simulink model "sliding_car"  (R2017a)
settings: Solver=VariableStepAuto  StartTime=0.0  StopTime=tf  RelTol=1e-3
values from neighbouring files (symbols this model uses):
  a = double(perc*D)    [init_vars.m]
  Cp_1 = 0    [init_vars.m]
  Cp_2 = 0    [init_vars.m]
  Fz_1 = g*(mc/4 + mi)    [init_vars.m]
  Fz_2 = g*(mc/4 + mi)    [init_vars.m]
  mu_1 = 1e-3    (= 0.001)    [init_vars.m]
  mu_2 = 1e-3    (= 0.001)    [init_vars.m]
  x0 = double(subs([qs; ps], [sys.descrip.syms.'; delta_i],                   [sys.descrip.model_params.'; delta_i_num]))    [init_vars.m]    (also in sim_blockdiagram.m)
undefined symbols (not defined in the file or in its folder): g, Ic_33, Ii_11, Ii_21, Ii_22, Ii_31, Ii_32, Ii_33, Il_11, Il_21, Il_22, Il_31, Il_32, Il_33, Io_11, Io_21, Io_22, Io_31, Io_32, Io_33, Ir_11, Ir_21, Ir_22, Ir_31, Ir_32, Ir_33, L, Lc, mc, mi, ml, mo, mr, R, sys, w
(part 2 of 5)

== matlab function sliding_car/Vehicle/Steering automobile model/Auxiliary matrices/Q ==
  data: x input; qp input; u input; kappa_1 input; kappa_2 input; alpha_1 input; alpha_2 input; Ii_11 parameter; Ii_21 parameter; Ii_22 parameter; Ii_31 parameter; Ii_32 parameter; Ii_33 parameter; Il_11 parameter; Il_21 parameter; Il_22 parameter; Il_31 parameter; Il_32 parameter; Il_33 parameter; Io_11 parameter; Io_21 parameter; Io_22 parameter; Io_31 parameter; Io_32 parameter; Io_33 parameter; Ir_11 parameter; Ir_21 parameter; Ir_22 parameter; Ir_31 parameter; Ir_32 parameter; Ir_33 parameter; Lc parameter; mc parameter; mi parameter; ml parameter; mo parameter; mr parameter; L parameter; w parameter; Q output
function Q  = InputMatrix(x, qp, u, kappa_1, kappa_2, alpha_1, alpha_2, ...
                          Ii_11, Ii_21, Ii_22, Ii_31, Ii_32, Ii_33, ...
                          Il_11, Il_21, Il_22, Il_31, Il_32, Il_33, ...
                          Io_11, Io_21, Io_22, Io_31, Io_32, Io_33, ...
                          Ir_11, Ir_21, Ir_22, Ir_31, Ir_32, Ir_33, ...
                          Lc, mc, mi, ml, mo, mr, L, w)
    %INPUTMATRIX
    %    Q = INPUTMATRIX(II_11,II_21,II_22,II_31,II_32,II_33,IL_11,IL_21,IL_22,IL_31,IL_32,IL_33,IO_11,IO_21,IO_22,IO_31,IO_32,IO_33,IR_11,IR_21,IR_22,IR_31,IR_32,IR_33,L,LC,DELTA_I,DELTA_O,DELTAP_I,DELTAP_O,F_PHI_I,F_PHI_L,F_PHI_O,F_PHI_R,MC,MI,ML,MO,MR,PHI_I,PHI_L,PHI_O,PHI_R,PHIP_I,PHIP_L,PHIP_O,PHIP_R,THETAP,THETA,W)

    %    This function was generated by the Symbolic Math Toolbox version 7.2.
    %    16-Oct-2020 13:53:49

    x_pos =  x(1);
    y_pos =  x(2);
    theta =  x(3);

    delta_i = x(4);
    delta_o = x(5);

    phi_i = x(6);
    phi_l = x(7);
    phi_o = x(8);
    phi_r = x(9);
    
    p1 = x(10);
    p2 = x(11);
    p3 = x(12);
    
    xp = qp(1);
    yp = qp(2);
    thetap = qp(3);
    deltap_i = qp(4);
    deltap_o = qp(5);
    phip_i = qp(6);
    phip_o = qp(7);
    phip_r = qp(8);
    phip_l = qp(9);
    
    f_phi_i = u(1);
    f_phi_o = u(2);
    f_phi_r = u(3);
    f_phi_l = u(4);

    
    t2 = sin(theta);
    t3 = cos(theta);
    t4 = thetap.^2;
    t5 = deltap_i.^2;
    t6 = delta_i+theta;
    t7 = sin(t6);
    t8 = deltap_o.^2;
    t9 = delta_o+theta;
    t10 = sin(t9);
    t11 = phi_l+theta;
    t12 = cos(t11);
    t13 = phi_r+theta;
    t14 = cos(t13);
    t15 = phip_l.^2;
    t16 = sin(t11);
    t17 = phip_r.^2;
    t18 = sin(t13);
    t19 = theta.*2.0;
    t20 = delta_i.*2.0;
    t21 = phi_i+t19+t20;
    t22 = cos(t21);
    t23 = phip_i.^2;
    t24 = delta_o.*2.0;
    t25 = phi_o+t19+t24;
    t26 = cos(t25);
    t27 = phip_o.^2;
    t28 = sin(t21);
    t29 = sin(t25);
    t30 = phi_l-t19;
    t31 = cos(t30);
    t32 = phi_l+t19;
    t33 = cos(t32);
    t34 = phi_r-t19;
    t35 = cos(t34);
    t36 = phi_r+t19;
    t37 = cos(t36);
    t38 = phi_l-theta;
    t39 = cos(t38);
    t40 = phi_l.*3.0;
    t41 = t40+theta;
    t42 = cos(t41);
    t43 = phi_r-theta;
    t44 = cos(t43);
    t45 = phi_r.*3.0;
    t46 = t45+theta;
    t47 = cos(t46);
    t48 = delta_i+phi_i+theta;
    t49 = cos(t48);
    t50 = delta_o+phi_o+theta;
    t51 = cos(t50);
    t52 = sin(t30);
    t53 = sin(t32);
    t54 = phi_l.*2.0;
    t55 = t54+theta;
    t56 = sin(t38);
    t57 = sin(t41);
    t58 = sin(t34);
    t59 = sin(t36);
    t60 = phi_r.*2.0;
    t61 = t60+theta;
    t62 = sin(t43);
    t63 = sin(t46);
    t64 = phi_l.*4.0;
    t65 = t64+theta;
    t66 = sin(t65);
    t67 = phi_r.*4.0;
    t68 = t67+theta;
    t69 = sin(t68);
    t70 = sin(t48);
    t71 = sin(t50);
    t72 = -phi_i+t19+t20;
    t73 = cos(t72);
    t74 = phi_i.*2.0;
    t75 = t19+t20+t74;
    t76 = cos(t75);
    t77 = t19+t20-t74;
    t78 = cos(t77);
    t79 = phi_i.*3.0;
    t80 = t19+t20+t79;
    t81 = cos(t80);
    t82 = -phi_o+t19+t24;
    t83 = cos(t82);
    t84 = phi_o.*2.0;
    t85 = t19+t24+t84;
    t86 = cos(t85);
    t87 = t19+t24-t84;
    t88 = cos(t87);
    t89 = phi_o.*3.0;
    t90 = t19+t24+t89;
    t91 = cos(t90);
    t92 = phi_i.*4.0;
    t93 = t19+t20+t92;
    t94 = t19+t20-t79;
    t95 = sin(t77);
    t96 = sin(t75);
    t97 = t19+t20-t92;
    t98 = sin(t97);
    t99 = sin(t93);
    t100 = phi_o.*4.0;
    t101 = t19+t24+t100;
    t102 = t19+t24-t89;
    t103 = sin(t87);
    t104 = sin(t85);
    t105 = t19+t24-t100;
    t106 = sin(t105);
    t107 = sin(t101);
    t108 = cos(t94);
    t109 = cos(t93);
    t110 = cos(t102);
    t111 = cos(t101);
    t112 = sin(t72);
    t113 = sin(t94);
    t114 = sin(t80);
    t115 = sin(t82);
    t116 = sin(t102);
    t117 = sin(t90);
    t118 = sin(t19);
    t119 = t19+t20;
    t120 = sin(t119);
    t121 = t19+t24;
    t122 = sin(t121);
    t123 = -t19+t54;
    t124 = cos(t123);
    t125 = t19+t54;
    t126 = cos(t125);
    t127 = -t19+t60;
    t128 = cos(t127);
    t129 = t19+t60;
    t130 = cos(t129);
    t131 = t40-theta;
    t132 = cos(t131);
    t133 = -t19+t40;
    t134 = cos(t133);
    t135 = t19+t40;
    t136 = cos(t135);
    t137 = t45-theta;
    t138 = cos(t137);
    t139 = -t19+t45;
    t140 = cos(t139);
    t141 = t19+t45;
    t142 = cos(t141);
    t143 = delta_i-phi_i+theta;
    t144 = cos(t143);
    t145 = delta_i-t79+theta;
    t146 = cos(t145);
    t147 = delta_i+t79+theta;
    t148 = cos(t147);
    t149 = delta_o-phi_o+theta;
    t150 = cos(t149);
    t151 = delta_o-t89+theta;
    t152 = cos(t151);
    t153 = delta_o+t89+theta;
    t154 = cos(t153);
    t155 = delta_i-t92+theta;
    t156 = delta_i+t92+theta;
    t157 = sin(t155);
    t158 = sin(t156);
    t159 = delta_o-t100+theta;
    t160 = delta_o+t100+theta;
    t161 = sin(t159);
    t162 = sin(t160);
    t163 = cos(t155);
    t164 = cos(t156);
    t165 = cos(t159);
    t166 = cos(t160);
    t167 = t54-theta;
    t168 = sin(t123);
    t169 = sin(t125);
    t170 = sin(t131);
    t171 = sin(t133);
    t172 = sin(t135);
    t173 = t60-theta;
    t174 = sin(t127);
    t175 = sin(t129);
    t176 = sin(t137);
    t177 = sin(t139);
    t178 = sin(t141);
    t179 = t64-theta;
    t180 = -t19+t64;
    t181 = t19+t64;
    t182 = sin(t179);
    t183 = sin(t180);
    t184 = sin(t181);
    t185 = t67-theta;
    t186 = -t19+t67;
    t187 = t19+t67;
    t188 = sin(t185);
    t189 = sin(t186);
    t190 = sin(t187);
    t191 = sin(t143);
    t192 = sin(t145);
    t193 = sin(t147);
    t194 = delta_i-t74+theta;
    t195 = delta_i+t74+theta;
    t196 = sin(t149);
    t197 = sin(t151);
    t198 = sin(t153);
    t199 = delta_o-t84+theta;
    t200 = delta_o+t84+theta;
    t201 = cos(t65);
    t202 = cos(t68);
    t203 = cos(t97);
    t204 = cos(t105);
    t205 = sin(t74);
    t206 = sin(t92);
    t207 = sin(t84);
    t208 = sin(t100);
    t209 = cos(t74);
    t210 = cos(t92);
    t211 = cos(t84);
    t212 = cos(t100);
    t213 = sin(t54);
    t214 = sin(t64);
    t215 = sin(t60);
    t216 = sin(t67);
    t217 = cos(t179);
    t218 = cos(t180);
    t219 = cos(t181);
    t220 = cos(t185);
    t221 = cos(t186);
    t222 = cos(t187);
    t223 = Ii_11.*t5.*t7.*(1.0./8.0);
    t224 = Ii_11.*t4.*t7.*(1.0./8.0);
    t225 = Ii_21.*t5.*t22.*(1.0./8.0);
    t226 = Ii_21.*t22.*t23.*(1.0./2.0);
    t227 = Ii_31.*t22.*t23.*(1.0./8.0);
    t228 = Ii_32.*t5.*t28.*(3.0./8.0);
    t229 = Ii_21.*t4.*t22.*(1.0./8.0);
    t230 = Ii_11.*t23.*t28.*(1.0./1.6e1);
    t231 = Ii_32.*t23.*t28.*(1.0./2.0);
    t232 = Ii_33.*t23.*t28.*(3.0./1.6e1);
    t233 = Ii_32.*t4.*t28.*(3.0./8.0);
    t234 = Ii_21.*t5.*t49.*(1.0./8.0);
    t235 = Ii_21.*t4.*t49.*(1.0./8.0);
    t236 = Ii_11.*t23.*t70.*(1.0./8.0);
    t237 = Ii_21.*t5.*t73.*(1.0./8.0);
    t238 = Ii_31.*t5.*t109.*(1.0./1.6e1);
    t239 = Ii_21.*t23.*t73.*(1.0./2.0);
    t240 = Ii_21.*t23.*t78.*(1.0./2.0);
    t241 = Ii_21.*t23.*t76.*(1.0./2.0);
    t242 = Ii_31.*t23.*t78.*(1.0./4.0);
    t243 = Ii_31.*t23.*t108.*(3.0./8.0);
    t244 = Ii_22.*t5.*t95.*(1.0./8.0);
    t245 = Ii_22.*t5.*t96.*(1.0./8.0);
    t246 = Ii_32.*t5.*t113.*(1.0./8.0);
    t247 = Ii_33.*t5.*t98.*(1.0./3.2e1);
    t248 = Ii_33.*t5.*t99.*(1.0./3.2e1);
    t249 = Ii_21.*t4.*t73.*(1.0./8.0);
    t250 = Ii_31.*t4.*t78.*(1.0./8.0);
    t251 = Ii_31.*t4.*t109.*(1.0./1.6e1);
    t252 = Ii_11.*t23.*t112.*(1.0./1.6e1);
    t253 = Ii_11.*t23.*t95.*(1.0./8.0);
    t254 = Ii_11.*t23.*t96.*(1.0./8.0);
    t255 = Ii_11.*t23.*t113.*(3.0./1.6e1);
    t256 = Ii_11.*t23.*t114.*(3.0./1.6e1);
    t257 = Ii_32.*t23.*t96.*(1.0./2.0);
    t258 = Ii_33.*t23.*t112.*(3.0./1.6e1);
    t259 = Ii_22.*t4.*t95.*(1.0./8.0);
    t260 = Ii_22.*t4.*t96.*(1.0./8.0);
    t261 = Ii_32.*t4.*t113.*(1.0./8.0);
    t262 = Ii_33.*t4.*t98.*(1.0./3.2e1);
    t263 = Ii_33.*t4.*t99.*(1.0./3.2e1);
    t264 = Ii_11.*t5.*t120.*(1.0./1.6e1);
    t265 = Ii_33.*t5.*t120.*(3.0./1.6e1);
    t266 = Ii_21.*t5.*t144.*(1.0./8.0);
    t267 = Ii_31.*t5.*t164.*(1.0./8.0);
    t268 = Ii_11.*t23.*t120.*(1.0./4.0);
    t269 = Ii_33.*t23.*t120.*(1.0./4.0);
    t270 = cos(t194);
    t271 = Ii_21.*t23.*t270.*(1.0./2.0);
    t272 = cos(t195);
    t273 = Ii_21.*t23.*t272.*(1.0./2.0);
    t274 = Ii_31.*t23.*t144.*(1.0./4.0);
    t275 = Ii_31.*t23.*t146.*(3.0./4.0);
    t276 = Ii_11.*t4.*t120.*(1.0./1.6e1);
    t277 = Ii_33.*t4.*t120.*(3.0./1.6e1);
    t278 = Ii_32.*t5.*t191.*(1.0./8.0);
    t279 = Ii_32.*t5.*t192.*(1.0./8.0);
    t280 = Ii_33.*t5.*t157.*(1.0./1.6e1);
    t281 = Ii_33.*t5.*t158.*(1.0./1.6e1);
    t282 = Ii_21.*t4.*t144.*(1.0./8.0);
    t283 = Ii_31.*t4.*t164.*(1.0./8.0);
    t284 = Ii_11.*t23.*t191.*(1.0./8.0);
    t285 = Ii_11.*t23.*t192.*(3.0./8.0);
    t286 = Ii_11.*t23.*t193.*(3.0./8.0);
    t287 = sin(t194);
    t288 = sin(t195);
    t289 = Ii_32.*t23.*t288.*(1.0./2.0);
    t290 = Ii_32.*t4.*t191.*(1.0./8.0);
    t291 = Ii_32.*t4.*t192.*(1.0./8.0);
    t292 = Ii_33.*t4.*t157.*(1.0./1.6e1);
    t293 = Ii_33.*t4.*t158.*(1.0./1.6e1);
    t294 = Ii_11.*phip_i.*t157.*thetap.*(1.0./2.0);
    t295 = Ii_33.*phip_i.*t158.*thetap.*(1.0./2.0);
    t296 = Ii_11.*deltap_i.*t7.*thetap.*(1.0./4.0);
    t297 = Ii_21.*deltap_i.*phip_i.*t22.*(1.0./8.0);
    t298 = Ii_21.*deltap_i.*t22.*thetap.*(1.0./4.0);
    t299 = Ii_32.*deltap_i.*phip_i.*t28.*(3.0./8.0);
    t300 = Ii_21.*phip_i.*t22.*thetap.*(1.0./8.0);
    t301 = Ii_32.*deltap_i.*t28.*thetap.*(3.0./4.0);
    t302 = Ii_32.*phip_i.*t28.*thetap.*(3.0./8.0);
    t303 = Ii_21.*deltap_i.*phip_i.*t49.*(1.0./4.0);
    t304 = Ii_21.*deltap_i.*t49.*thetap.*(1.0./4.0);
    t305 = Ii_21.*phip_i.*t49.*thetap.*(1.0./4.0);
    t306 = Ii_21.*deltap_i.*phip_i.*t108.*(3.0./8.0);
    t307 = Ii_31.*deltap_i.*phip_i.*t203.*(1.0./4.0);
    t308 = Ii_31.*deltap_i.*phip_i.*t109.*(1.0./4.0);
    t309 = Ii_21.*deltap_i.*t73.*thetap.*(1.0./4.0);
    t310 = Ii_31.*deltap_i.*t78.*thetap.*(1.0./4.0);
    t311 = Ii_31.*deltap_i.*t109.*thetap.*(1.0./8.0);
    t312 = Ii_31.*deltap_i.*phip_i.*t209.*(1.0./2.0);
    t313 = Ii_31.*deltap_i.*phip_i.*t210.*(3.0./2.0);
    t314 = Ii_11.*deltap_i.*phip_i.*t98.*(1.0./8.0);
    t315 = Ii_22.*deltap_i.*phip_i.*t96.*(1.0./4.0);
    t316 = Ii_32.*deltap_i.*phip_i.*t112.*(3.0./8.0);
    t317 = Ii_33.*deltap_i.*phip_i.*t95.*(1.0./4.0);
    t318 = Ii_33.*deltap_i.*phip_i.*t99.*(1.0./8.0);
    t319 = Ii_21.*phip_i.*t108.*thetap.*(3.0./8.0);
    t320 = Ii_31.*phip_i.*t203.*thetap.*(1.0./4.0);
    t321 = Ii_31.*phip_i.*t109.*thetap.*(1.0./4.0);
    t322 = Ii_22.*deltap_i.*t95.*thetap.*(1.0./4.0);
    t323 = Ii_22.*deltap_i.*t96.*thetap.*(1.0./4.0);
    t324 = Ii_32.*deltap_i.*t113.*thetap.*(1.0./4.0);
    t325 = Ii_33.*deltap_i.*t98.*thetap.*(1.0./1.6e1);
    t326 = Ii_33.*deltap_i.*t99.*thetap.*(1.0./1.6e1);
    t327 = Ii_33.*deltap_i.*phip_i.*t205.*(1.0./2.0);
    t328 = Ii_33.*deltap_i.*phip_i.*t206.*(3.0./4.0);
    t329 = Ii_31.*phip_i.*t209.*thetap.*(1.0./2.0);
    t330 = Ii_31.*phip_i.*t210.*thetap.*(3.0./2.0);
    t331 = Ii_11.*phip_i.*t98.*thetap.*(1.0./8.0);
    t332 = Ii_22.*phip_i.*t96.*thetap.*(1.0./4.0);
    t333 = Ii_32.*phip_i.*t112.*thetap.*(3.0./8.0);
    t334 = Ii_33.*phip_i.*t95.*thetap.*(1.0./4.0);
    t335 = Ii_33.*phip_i.*t99.*thetap.*(1.0./8.0);
    t336 = Ii_33.*phip_i.*t205.*thetap.*(1.0./2.0);
    t337 = Ii_33.*phip_i.*t206.*thetap.*(3.0./4.0);
    t338 = Ii_21.*deltap_i.*phip_i.*t146.*(3.0./4.0);
    t339 = Ii_31.*deltap_i.*phip_i.*t163;
    t340 = Ii_31.*deltap_i.*phip_i.*t164;
    t341 = Ii_11.*deltap_i.*t120.*thetap.*(1.0./8.0);
    t342 = Ii_33.*deltap_i.*t120.*thetap.*(3.0./8.0);
    t343 = Ii_21.*deltap_i.*t144.*thetap.*(1.0./4.0);
    t344 = Ii_31.*deltap_i.*t164.*thetap.*(1.0./4.0);
    t345 = Ii_11.*deltap_i.*phip_i.*t157.*(1.0./2.0);
    t346 = Ii_33.*deltap_i.*phip_i.*t158.*(1.0./2.0);
    t347 = Ii_21.*phip_i.*t146.*thetap.*(3.0./4.0);
    t348 = Ii_31.*phip_i.*t163.*thetap;
    t349 = Ii_31.*phip_i.*t164.*thetap;
    t350 = Ii_32.*deltap_i.*t191.*thetap.*(1.0./4.0);
    t351 = Ii_32.*deltap_i.*t192.*thetap.*(1.0./4.0);
    t352 = Ii_33.*deltap_i.*t157.*thetap.*(1.0./8.0);
    t353 = Ii_33.*deltap_i.*t158.*thetap.*(1.0./8.0);
    t354 = Io_11.*t8.*t10.*(1.0./8.0);
    t355 = Io_11.*t4.*t10.*(1.0./8.0);
    t356 = Io_21.*t8.*t26.*(1.0./8.0);
    t357 = Io_21.*t26.*t27.*(1.0./2.0);
    t358 = Io_31.*t26.*t27.*(1.0./8.0);
    t359 = Io_32.*t8.*t29.*(3.0./8.0);
    t360 = Io_21.*t4.*t26.*(1.0./8.0);
    t361 = Io_11.*t27.*t29.*(1.0./1.6e1);
    t362 = Io_32.*t27.*t29.*(1.0./2.0);
    t363 = Io_33.*t27.*t29.*(3.0./1.6e1);
    t364 = Io_32.*t4.*t29.*(3.0./8.0);
    t365 = Io_21.*t8.*t51.*(1.0./8.0);
    t366 = Io_21.*t4.*t51.*(1.0./8.0);
    t367 = Io_11.*t27.*t71.*(1.0./8.0);
    t368 = Io_21.*t8.*t83.*(1.0./8.0);
    t369 = Io_31.*t8.*t111.*(1.0./1.6e1);
    t370 = Io_21.*t27.*t83.*(1.0./2.0);
    t371 = Io_21.*t27.*t88.*(1.0./2.0);
    t372 = Io_21.*t27.*t86.*(1.0./2.0);
    t373 = Io_31.*t27.*t88.*(1.0./4.0);
    t374 = Io_31.*t27.*t110.*(3.0./8.0);
    t375 = Io_22.*t8.*t103.*(1.0./8.0);
    t376 = Io_22.*t8.*t104.*(1.0./8.0);
    t377 = Io_32.*t8.*t116.*(1.0./8.0);
    t378 = Io_33.*t8.*t106.*(1.0./3.2e1);
    t379 = Io_33.*t8.*t107.*(1.0./3.2e1);
    t380 = Io_21.*t4.*t83.*(1.0./8.0);
    t381 = Io_31.*t4.*t88.*(1.0./8.0);
    t382 = Io_31.*t4.*t111.*(1.0./1.6e1);
    t383 = Io_11.*t27.*t115.*(1.0./1.6e1);
    t384 = Io_11.*t27.*t103.*(1.0./8.0);
    t385 = Io_11.*t27.*t104.*(1.0./8.0);
    t386 = Io_11.*t27.*t116.*(3.0./1.6e1);
    t387 = Io_11.*t27.*t117.*(3.0./1.6e1);
    t388 = Io_32.*t27.*t104.*(1.0./2.0);
    t389 = Io_33.*t27.*t115.*(3.0./1.6e1);
    t390 = Io_22.*t4.*t103.*(1.0./8.0);
    t391 = Io_22.*t4.*t104.*(1.0./8.0);
    t392 = Io_32.*t4.*t116.*(1.0./8.0);
    t393 = Io_33.*t4.*t106.*(1.0./3.2e1);
    t394 = Io_33.*t4.*t107.*(1.0./3.2e1);
    t395 = Io_11.*t8.*t122.*(1.0./1.6e1);
    t396 = Io_33.*t8.*t122.*(3.0./1.6e1);
    t397 = Io_21.*t8.*t150.*(1.0./8.0);
    t398 = Io_31.*t8.*t166.*(1.0./8.0);
    t399 = Io_11.*t27.*t122.*(1.0./4.0);
    t400 = Io_33.*t27.*t122.*(1.0./4.0);
    t401 = cos(t199);
    t402 = Io_21.*t27.*t401.*(1.0./2.0);
    t403 = cos(t200);
    t404 = Io_21.*t27.*t403.*(1.0./2.0);
    t405 = Io_31.*t27.*t150.*(1.0./4.0);
    t406 = Io_31.*t27.*t152.*(3.0./4.0);
    t407 = Io_11.*t4.*t122.*(1.0./1.6e1);
    t408 = Io_33.*t4.*t122.*(3.0./1.6e1);
    t409 = Io_32.*t8.*t196.*(1.0./8.0);
    t410 = Io_32.*t8.*t197.*(1.0./8.0);
    t411 = Io_33.*t8.*t161.*(1.0./1.6e1);
    t412 = Io_33.*t8.*t162.*(1.0./1.6e1);
    t413 = Io_21.*t4.*t150.*(1.0./8.0);
    t414 = Io_31.*t4.*t166.*(1.0./8.0);
    t415 = Io_11.*t27.*t196.*(1.0./8.0);
    t416 = Io_11.*t27.*t197.*(3.0./8.0);
    t417 = Io_11.*t27.*t198.*(3.0./8.0);
    t418 = sin(t199);
    t419 = sin(t200);
    t420 = Io_32.*t27.*t419.*(1.0./2.0);
    t421 = Io_32.*t4.*t196.*(1.0./8.0);
    t422 = Io_32.*t4.*t197.*(1.0./8.0);
    t423 = Io_33.*t4.*t161.*(1.0./1.6e1);
    t424 = Io_33.*t4.*t162.*(1.0./1.6e1);
    t425 = Io_11.*phip_o.*t161.*thetap.*(1.0./2.0);
    t426 = Io_33.*phip_o.*t162.*thetap.*(1.0./2.0);
    t427 = Io_11.*deltap_o.*t10.*thetap.*(1.0./4.0);
    t428 = Io_21.*deltap_o.*phip_o.*t26.*(1.0./8.0);
    t429 = Io_21.*deltap_o.*t26.*thetap.*(1.0./4.0);
    t430 = Io_32.*deltap_o.*phip_o.*t29.*(3.0./8.0);
    t431 = Io_21.*phip_o.*t26.*thetap.*(1.0./8.0);
    t432 = Io_32.*deltap_o.*t29.*thetap.*(3.0./4.0);
    t433 = Io_32.*phip_o.*t29.*thetap.*(3.0./8.0);
    t434 = Io_21.*deltap_o.*phip_o.*t51.*(1.0./4.0);
    t435 = Io_21.*deltap_o.*t51.*thetap.*(1.0./4.0);
    t436 = Io_21.*phip_o.*t51.*thetap.*(1.0./4.0);
    t437 = Io_21.*deltap_o.*phip_o.*t110.*(3.0./8.0);
    t438 = Io_31.*deltap_o.*phip_o.*t204.*(1.0./4.0);
    t439 = Io_31.*deltap_o.*phip_o.*t111.*(1.0./4.0);
    t440 = Io_21.*deltap_o.*t83.*thetap.*(1.0./4.0);
    t441 = Io_31.*deltap_o.*t88.*thetap.*(1.0./4.0);
    t442 = Io_31.*deltap_o.*t111.*thetap.*(1.0./8.0);
    t443 = Io_31.*deltap_o.*phip_o.*t211.*(1.0./2.0);
    t444 = Io_31.*deltap_o.*phip_o.*t212.*(3.0./2.0);
    t445 = Io_11.*deltap_o.*phip_o.*t106.*(1.0./8.0);
    t446 = Io_22.*deltap_o.*phip_o.*t104.*(1.0./4.0);
    t447 = Io_32.*deltap_o.*phip_o.*t115.*(3.0./8.0);
    t448 = Io_33.*deltap_o.*phip_o.*t103.*(1.0./4.0);
    t449 = Io_33.*deltap_o.*phip_o.*t107.*(1.0./8.0);
    t450 = Io_21.*phip_o.*t110.*thetap.*(3.0./8.0);
    t451 = Io_31.*phip_o.*t204.*thetap.*(1.0./4.0);
    t452 = Io_31.*phip_o.*t111.*thetap.*(1.0./4.0);
    t453 = Io_22.*deltap_o.*t103.*thetap.*(1.0./4.0);
    t454 = Io_22.*deltap_o.*t104.*thetap.*(1.0./4.0);
    t455 = Io_32.*deltap_o.*t116.*thetap.*(1.0./4.0);
    t456 = Io_33.*deltap_o.*t106.*thetap.*(1.0./1.6e1);
    t457 = Io_33.*deltap_o.*t107.*thetap.*(1.0./1.6e1);
    t458 = Io_33.*deltap_o.*phip_o.*t207.*(1.0./2.0);
    t459 = Io_33.*deltap_o.*phip_o.*t208.*(3.0./4.0);
    t460 = Io_31.*phip_o.*t211.*thetap.*(1.0./2.0);
    t461 = Io_31.*phip_o.*t212.*thetap.*(3.0./2.0);
    t462 = Io_11.*phip_o.*t106.*thetap.*(1.0./8.0);
    t463 = Io_22.*phip_o.*t104.*thetap.*(1.0./4.0);
    t464 = Io_32.*phip_o.*t115.*thetap.*(3.0./8.0);
    t465 = Io_33.*phip_o.*t103.*thetap.*(1.0./4.0);
    t466 = Io_33.*phip_o.*t107.*thetap.*(1.0./8.0);
    t467 = Io_33.*phip_o.*t207.*thetap.*(1.0./2.0);
    t468 = Io_33.*phip_o.*t208.*thetap.*(3.0./4.0);
    t469 = Io_21.*deltap_o.*phip_o.*t152.*(3.0./4.0);
    t470 = Io_31.*deltap_o.*phip_o.*t165;
    t471 = Io_31.*deltap_o.*phip_o.*t166;
    t472 = Io_11.*deltap_o.*t122.*thetap.*(1.0./8.0);
    t473 = Io_33.*deltap_o.*t122.*thetap.*(3.0./8.0);
    t474 = Io_21.*deltap_o.*t150.*thetap.*(1.0./4.0);
    t475 = Io_31.*deltap_o.*t166.*thetap.*(1.0./4.0);
    t476 = Io_11.*deltap_o.*phip_o.*t161.*(1.0./2.0);
    t477 = Io_33.*deltap_o.*phip_o.*t162.*(1.0./2.0);
    t478 = Io_21.*phip_o.*t152.*thetap.*(3.0./4.0);
    t479 = Io_31.*phip_o.*t165.*thetap;
    t480 = Io_31.*phip_o.*t166.*thetap;
    t481 = Io_32.*deltap_o.*t196.*thetap.*(1.0./4.0);
    t482 = Io_32.*deltap_o.*t197.*thetap.*(1.0./4.0);
    t483 = Io_33.*deltap_o.*t161.*thetap.*(1.0./8.0);
    t484 = Io_33.*deltap_o.*t162.*thetap.*(1.0./8.0);
    t485 = cos(delta_i);
    t486 = sin(delta_i);
    t487 = cos(t20);
    t488 = sin(t20);
    t489 = cos(t19);
    t490 = sin(phi_i);
    t491 = cos(phi_i);
    t492 = cos(t79);
    t493 = sin(t79);
    t494 = cos(delta_o);
    t495 = sin(delta_o);
    t496 = cos(t24);
    t497 = sin(t24);
    t498 = sin(phi_o);
    t499 = cos(phi_o);
    t500 = cos(t89);
    t501 = sin(t89);
    t502 = cos(phi_r);
    t503 = t502.^2;
    t504 = sin(phi_r);
    t505 = t504.^2;
    t506 = t2.^2;
    t507 = t503.^2;
    t508 = t3.^2;
    t509 = t505.^2;
    t510 = cos(phi_l);
    t511 = t510.^2;
    t512 = sin(phi_l);
    t513 = t512.^2;
    t514 = t511.^2;
    t515 = t513.^2;
    aux = t223+t224+t225+t226+t227+t228+t229+t230+t231+t232+t233+t234+t235+t236+t237+t238+t239+t240+t241+t242+t243+...
         t244+t245+t246+t247+t248+t249+t250+t251+t252+t253+t254+t255+t256+t257+t258+t259+t260+t261+t262+t263+t264+...
         t265+t266+t267+t268+t269+t271+t273+t274+t275+t276+t277+t278+t279+t280+t281+t282+t283+t284+t285+t286+t289+...
         t290+t291+t292+t293+t294+t295+t296+t297+t298+t299+t300+t301+t302+t303+t304+t305+t306+t307+t308+t309+t310+...
         t311+t312+t313+t314+t315+t316+t317+t318+t319+t320+t321+t322+t323+t324+t325+t326+t327+t328+t329+t330+t331+...
         t332+t333+t334+t335+t336+t337+t338+t339+t340+t341+t342+t343+t344+t345+t346+t347+t348+t349+t350+t351+t352+...
         t353+t354+t355+t356+t357+t358+t359+t360+t361+t362+t363+t364+t365+t366+t367+t368+t369+t370+t371+t372+t373+...
         t374+t375+t376+t377+t378+t379+t380+t381+t382+t383+t384+t385+t386+t387+t388+t389+t390+t391+t392+t393+t394+...
         t395+t396+t397+t398+t399+t400+t402+t404+t405+t406+t407+t408+t409+t410+t411+t412+t413+t414+t415+t416+t417+...
         t420+t421+t422+t423+t424+t425+t426+t427+t428+t429+t430+t431+t432+t433+t434+t435+t436+t437+t438+t439+t440+...
         t441+t442+t443+t444+t445+t446+t447+t448+t449+t450+t451+t452+t453+t454+t455+t456+t457+t458+t459+t460+t461+...
         t462+t463+t464+t465+t466+t467+t468+t469+t470+t471+t472+t473+t474+t475+t476+t477+t478+t479+t480+t481+t482;
     
    aux2 = t354+t355+t356+t357+t358+t359+t360+t361+t362+t363+t364+t365+t366+t367+t368+t369+t370+t371+t372+t373+t374+...
           t375+t376+t377+t378+t379+t380+t381+t382+t383+t384+t385+t386+t387+t388+t389+t390+t391+t392+t393+t394+t395+...
           t396+t397+t398+t399+t400+t402+t404+t405+t406+t407+t408+t409+t410+t411+t412+t413+t414+t415+t416+t417+t420+...
           t421+t422+t423+t424+t425+t426+t427+t428+t429+t430+t431+t432+t433+t434+t435+t436+t437+t438+t439+t440+t441+...
           t442+t443+t444+t445+t446+t447+t448+t449+t450+t451+t452+t453+t454+t455+t456+t457+t458+t459+t460+t461+t462+...
           t463+t464+t465+t466+t467+t468+t469+t470+t471+t472+t473+t474+t475+t476+t477+t478+t479+t480+t481+t482+t483+t484;
    
    aux3 = t223+t224+t225+t226+t227+t228+t229+t230+t231+t232+t233+t234+t235+t236+t237+t238+t239+t240+t241+t242+t243+...
           t244+t245+t246+t247+t248+t249+t250+t251+t252+t253+t254+t255+t256+t257+t258+t259+t260+t261+t262+t263+t264+...
           t265+t266+t267+t268+t269+t271+t273+t274+t275+t276+t277+t278+t279+t280+t281+t282+t283+t284+t285+t286+t289+t290+...
           t291+t292+t293+t294+t295+t296+t297+t298+t299+t300+t301+t302+t303+t304+t305+t306+t307+t308+t309+t310+t311+t312+...
           t313+t314+t315+t316+t317+t318+t319+t320+t321+t322+t323+t324+t325+t326+t327+t328+t329+t330+t331+t332+t333+...
           t334+t335+t336+t337+t338+t339+t340+t341+t342+t343+t344+t345+t346+t347+t348+t349+t350+t351+t352+t353;
    
    Q11 = t4.*(L.*mi.*t2.*2.0+L.*mo.*t2.*2.0+Lc.*mc.*t2.*2.0-mi.*t3.*w-ml.*t3.*w+mo.*t3.*w+mr.*t3.*w).*(-1.0./2.0);
    
    Q21 = t4.*(L.*mi.*t3.*2.0+L.*mo.*t3.*2.0+Lc.*mc.*t3.*2.0+mi.*t2.*w+ml.*t2.*w-mo.*t2.*w-mr.*t2.*w).*(1.0./2.0);
    
    Q31 = aux+t483+t484+Il_32.*t15.*sin(t55).*(1.0./2.0)+Il_32.*t15.*sin(t167).*(1.0./2.0)+Ir_32.*t17.*sin(t61).*(1.0./2.0)+...
         Ir_32.*t17.*sin(t173).*(1.0./2.0)-Ii_33.*t4.*t7.*(1.0./8.0)-Ii_33.*t5.*t7.*(1.0./8.0)-Ii_22.*t23.*t28.*(1.0./4.0)-...
         Ii_31.*t23.*t49.*(1.0./4.0)-Ii_21.*t4.*t81.*(1.0./8.0)-Ii_32.*t4.*t70.*(1.0./8.0)-Ii_21.*t5.*t81.*(1.0./8.0)-Ii_32.*t5.*t70.*(1.0./8.0)-...
         Ii_31.*t4.*t76.*(1.0./8.0)-Ii_31.*t5.*t76.*(1.0./8.0)-Ii_11.*t4.*t98.*(1.0./3.2e1)-Ii_11.*t4.*t99.*(1.0./3.2e1)-...
         Ii_11.*t5.*t98.*(1.0./3.2e1)-Ii_11.*t5.*t99.*(1.0./3.2e1)-Ii_33.*t23.*t70.*(1.0./8.0)-Ii_31.*t23.*t73.*(1.0./8.0)-...
         Ii_31.*t23.*t76.*(1.0./4.0)-Ii_33.*t4.*t95.*(1.0./8.0)-Ii_21.*t4.*t108.*(1.0./8.0)-Ii_33.*t4.*t96.*(1.0./8.0)-...
         Ii_33.*t5.*t95.*(1.0./8.0)-Ii_33.*t5.*t96.*(1.0./8.0)-Ii_31.*t23.*t81.*(3.0./8.0)-Ii_22.*t4.*t120.*(1.0./4.0)-...
         Ii_22.*t5.*t120.*(1.0./4.0)-Ii_32.*t4.*t112.*(3.0./8.0)-Ii_32.*t5.*t112.*(3.0./8.0)-Ii_32.*t4.*t114.*(1.0./8.0)-...
         Ii_32.*t23.*t95.*(1.0./2.0)-Ii_32.*t5.*t114.*(1.0./8.0)-Ii_33.*t23.*t95.*(1.0./8.0)-Ii_33.*t23.*t96.*(1.0./8.0)-...
         Ii_22.*t23.*t112.*(1.0./4.0)-Ii_22.*t23.*t120.*(1.0./2.0)-Ii_32.*t23.*t112.*(1.0./2.0)-Ii_33.*t23.*t113.*(3.0./1.6e1)-...
         Ii_33.*t23.*t114.*(3.0./1.6e1)-Ii_21.*t4.*t146.*(1.0./8.0)-Ii_11.*t4.*t157.*(1.0./1.6e1)-Ii_21.*t5.*t146.*(1.0./8.0)-...
         Ii_11.*t4.*t158.*(1.0./1.6e1)-Ii_11.*t5.*t157.*(1.0./1.6e1)-Ii_21.*t4.*t148.*(1.0./8.0)-Ii_11.*t5.*t158.*(1.0./1.6e1)-...
         Ii_21.*t5.*t148.*(1.0./8.0)-Ii_31.*t4.*t163.*(1.0./8.0)-Ii_31.*t5.*t163.*(1.0./8.0)-Ii_31.*t23.*t148.*(3.0./4.0)-Ii_32.*t4.*t193.*(1.0./8.0)-...
         Ii_32.*t5.*t193.*(1.0./8.0)-Ii_31.*t4.*t203.*(1.0./1.6e1)-Ii_33.*t23.*t191.*(1.0./8.0)-Ii_33.*t23.*t192.*(3.0./8.0)-Ii_33.*t23.*t193.*(3.0./8.0)-...
         Ii_32.*t23.*t287.*(1.0./2.0)+Il_11.*t2.*t4.*(1.0./8.0)+Il_21.*t4.*t12.*(1.0./8.0)-Il_33.*t2.*t4.*(1.0./8.0)+Il_11.*t15.*t16.*(1.0./8.0)-...
         Il_32.*t4.*t16.*(1.0./8.0)+Il_21.*t4.*t31.*(1.0./8.0)+Il_21.*t4.*t33.*(1.0./8.0)-Il_31.*t12.*t15.*(1.0./4.0)+Il_21.*t4.*t39.*(1.0./8.0)-Il_33.*t15.*t16.*(1.0./8.0)-...
         Il_21.*t4.*t42.*(1.0./8.0)+Il_21.*t15.*t31.*(1.0./2.0)+Il_21.*t15.*t33.*(1.0./2.0)-Il_31.*t15.*t31.*(1.0./8.0)-...
         Il_11.*t15.*t52.*(1.0./1.6e1)+Il_11.*t15.*t53.*(1.0./1.6e1)+Il_31.*t15.*t33.*(1.0./8.0)-Il_11.*t4.*t66.*(1.0./1.6e1)-...
         Il_11.*t15.*t56.*(1.0./8.0)+Il_11.*t15.*t57.*(3.0./8.0)+Il_31.*t15.*t39.*(1.0./4.0)-Il_31.*t15.*t42.*(3.0./4.0)+Il_32.*t4.*t52.*(3.0./8.0)+...
         Il_22.*t15.*t52.*(1.0./4.0)+Il_32.*t4.*t53.*(3.0./8.0)-Il_22.*t15.*t53.*(1.0./4.0)-Il_32.*t4.*t56.*(1.0./8.0)-Il_32.*t4.*t57.*(1.0./8.0)+...
         Il_32.*t15.*t52.*(1.0./2.0)+Il_32.*t15.*t53.*(1.0./2.0)-Il_33.*t15.*t52.*(3.0./1.6e1)+Il_33.*t15.*t53.*(3.0./1.6e1)+Il_33.*t4.*t66.*(1.0./1.6e1)+...
         Il_33.*t15.*t56.*(1.0./8.0)-Il_33.*t15.*t57.*(3.0./8.0)+Il_11.*t4.*t118.*(1.0./1.6e1)+Il_11.*t15.*t118.*(1.0./4.0)-Il_22.*t4.*t118.*(1.0./4.0)-...
         Il_22.*t15.*t118.*(1.0./2.0)+Il_33.*t4.*t118.*(3.0./1.6e1)-Il_21.*t4.*t132.*(1.0./8.0)-Il_21.*t4.*t134.*(1.0./8.0)+Il_31.*t4.*t124.*(1.0./8.0)+...
         Il_21.*t15.*t124.*(1.0./2.0)-Il_21.*t4.*t136.*(1.0./8.0)-Il_31.*t4.*t126.*(1.0./8.0)+Il_21.*t15.*t126.*(1.0./2.0)+Il_33.*t15.*t118.*(1.0./4.0)+...
         Il_31.*t15.*t124.*(1.0./4.0)-Il_31.*t15.*t126.*(1.0./4.0)+Il_31.*t15.*t132.*(3.0./4.0)+Il_31.*t15.*t134.*(3.0./8.0)-Il_31.*t15.*t136.*(3.0./8.0)-...
         Il_11.*t15.*t168.*(1.0./8.0)-Il_22.*t4.*t168.*(1.0./8.0)+Il_11.*t15.*t169.*(1.0./8.0)+Il_22.*t4.*t169.*(1.0./8.0)-Il_11.*t15.*t170.*(3.0./8.0)+...
         Il_11.*t4.*t182.*(1.0./1.6e1)-Il_11.*t15.*t171.*(3.0./1.6e1)+Il_11.*t4.*t183.*(1.0./3.2e1)+Il_11.*t15.*t172.*(3.0./1.6e1)-...
         Il_11.*t4.*t184.*(1.0./3.2e1)+Il_33.*t4.*t168.*(1.0./8.0)-Il_32.*t4.*t170.*(1.0./8.0)-Il_33.*t4.*t169.*(1.0./8.0)-Il_32.*t4.*t171.*(1.0./8.0)-...
         Il_32.*t4.*t172.*(1.0./8.0)+Il_32.*t15.*t168.*(1.0./2.0)+Il_32.*t15.*t169.*(1.0./2.0)+Il_33.*t15.*t168.*(1.0./8.0)-Il_33.*t15.*t169.*(1.0./8.0)+...
         Il_33.*t15.*t170.*(3.0./8.0)-Il_33.*t4.*t182.*(1.0./1.6e1)+Il_33.*t15.*t171.*(3.0./1.6e1)-Il_33.*t4.*t183.*(1.0./3.2e1)-Il_33.*t15.*t172.*(3.0./1.6e1)+...
         Il_33.*t4.*t184.*(1.0./3.2e1)+Il_31.*t4.*t201.*(1.0./8.0)-Il_31.*t4.*t217.*(1.0./8.0)-Il_31.*t4.*t218.*(1.0./1.6e1)+Il_31.*t4.*t219.*(1.0./1.6e1)-...
         Io_33.*t4.*t10.*(1.0./8.0)-Io_33.*t8.*t10.*(1.0./8.0)-Io_22.*t27.*t29.*(1.0./4.0)-Io_32.*t4.*t71.*(1.0./8.0)-Io_31.*t27.*t51.*(1.0./4.0)-...
         Io_32.*t8.*t71.*(1.0./8.0)-Io_21.*t4.*t91.*(1.0./8.0)-Io_21.*t8.*t91.*(1.0./8.0)-Io_11.*t4.*t106.*(1.0./3.2e1)-Io_31.*t4.*t86.*(1.0./8.0)-...
         Io_11.*t4.*t107.*(1.0./3.2e1)-Io_11.*t8.*t106.*(1.0./3.2e1)-Io_31.*t8.*t86.*(1.0./8.0)-Io_11.*t8.*t107.*(1.0./3.2e1)-Io_33.*t27.*t71.*(1.0./8.0)-...
         Io_21.*t4.*t110.*(1.0./8.0)-Io_33.*t4.*t103.*(1.0./8.0)-Io_31.*t27.*t83.*(1.0./8.0)-Io_33.*t4.*t104.*(1.0./8.0)-Io_31.*t27.*t86.*(1.0./4.0)-Io_33.*t8.*t103.*(1.0./8.0)-...
         Io_33.*t8.*t104.*(1.0./8.0)-Io_22.*t4.*t122.*(1.0./4.0)-Io_31.*t27.*t91.*(3.0./8.0)-Io_32.*t4.*t115.*(3.0./8.0)-Io_22.*t8.*t122.*(1.0./4.0)-...
         Io_32.*t4.*t117.*(1.0./8.0)-Io_32.*t8.*t115.*(3.0./8.0)-Io_32.*t8.*t117.*(1.0./8.0)-Io_32.*t27.*t103.*(1.0./2.0)-Io_33.*t27.*t103.*(1.0./8.0)-...
         Io_22.*t27.*t115.*(1.0./4.0)-Io_33.*t27.*t104.*(1.0./8.0)-Io_22.*t27.*t122.*(1.0./2.0)-Io_32.*t27.*t115.*(1.0./2.0)-Io_11.*t4.*t161.*(1.0./1.6e1)-...
         Io_33.*t27.*t116.*(3.0./1.6e1)-Io_11.*t4.*t162.*(1.0./1.6e1)-Io_21.*t4.*t152.*(1.0./8.0)-Io_33.*t27.*t117.*(3.0./1.6e1)-Io_21.*t4.*t154.*(1.0./8.0)-...
         Io_11.*t8.*t161.*(1.0./1.6e1)-Io_11.*t8.*t162.*(1.0./1.6e1)-Io_21.*t8.*t152.*(1.0./8.0)-Io_21.*t8.*t154.*(1.0./8.0)-Io_31.*t4.*t165.*(1.0./8.0)-...
         Io_31.*t8.*t165.*(1.0./8.0)-Io_31.*t27.*t154.*(3.0./4.0)-Io_32.*t4.*t198.*(1.0./8.0)-Io_32.*t8.*t198.*(1.0./8.0)-Io_31.*t4.*t204.*(1.0./1.6e1)-...
         Io_33.*t27.*t196.*(1.0./8.0)-Io_33.*t27.*t197.*(3.0./8.0)-Io_33.*t27.*t198.*(3.0./8.0)-Io_32.*t27.*t418.*(1.0./2.0)+Ir_11.*t2.*t4.*(1.0./8.0)+...
         Ir_21.*t4.*t14.*(1.0./8.0)-Ir_33.*t2.*t4.*(1.0./8.0)+Ir_11.*t17.*t18.*(1.0./8.0)-Ir_32.*t4.*t18.*(1.0./8.0)+Ir_21.*t4.*t35.*(1.0./8.0)+...
         Ir_21.*t4.*t37.*(1.0./8.0)-Ir_31.*t14.*t17.*(1.0./4.0)-Ir_33.*t17.*t18.*(1.0./8.0)+Ir_21.*t4.*t44.*(1.0./8.0)-Ir_21.*t4.*t47.*(1.0./8.0)+...
         Ir_21.*t17.*t35.*(1.0./2.0)+Ir_21.*t17.*t37.*(1.0./2.0)-Ir_31.*t17.*t35.*(1.0./8.0)-Ir_11.*t4.*t69.*(1.0./1.6e1)+Ir_31.*t17.*t37.*(1.0./8.0)-...
         Ir_11.*t17.*t58.*(1.0./1.6e1)+Ir_11.*t17.*t59.*(1.0./1.6e1)-Ir_11.*t17.*t62.*(1.0./8.0)+Ir_11.*t17.*t63.*(3.0./8.0)+Ir_31.*t17.*t44.*(1.0./4.0)+...
         Ir_32.*t4.*t58.*(3.0./8.0)-Ir_31.*t17.*t47.*(3.0./4.0)+Ir_32.*t4.*t59.*(3.0./8.0)+Ir_22.*t17.*t58.*(1.0./4.0)-Ir_22.*t17.*t59.*(1.0./4.0)-...
         Ir_32.*t4.*t62.*(1.0./8.0)-Ir_32.*t4.*t63.*(1.0./8.0)+Ir_33.*t4.*t69.*(1.0./1.6e1)+Ir_32.*t17.*t58.*(1.0./2.0)+Ir_32.*t17.*t59.*(1.0./2.0)-...
         Ir_33.*t17.*t58.*(3.0./1.6e1)+Ir_33.*t17.*t59.*(3.0./1.6e1)+Ir_33.*t17.*t62.*(1.0./8.0)-Ir_33.*t17.*t63.*(3.0./8.0)+Ir_11.*t4.*t118.*(1.0./1.6e1)-...
         Ir_22.*t4.*t118.*(1.0./4.0)+Ir_11.*t17.*t118.*(1.0./4.0)+Ir_33.*t4.*t118.*(3.0./1.6e1)-Ir_22.*t17.*t118.*(1.0./2.0)-Ir_21.*t4.*t138.*(1.0./8.0)+...
         Ir_31.*t4.*t128.*(1.0./8.0)-Ir_21.*t4.*t140.*(1.0./8.0)-Ir_31.*t4.*t130.*(1.0./8.0)+Ir_21.*t17.*t128.*(1.0./2.0)-Ir_21.*t4.*t142.*(1.0./8.0)+...
         Ir_21.*t17.*t130.*(1.0./2.0)+Ir_33.*t17.*t118.*(1.0./4.0)+Ir_31.*t17.*t128.*(1.0./4.0)-Ir_31.*t17.*t130.*(1.0./4.0)+Ir_31.*t17.*t138.*(3.0./4.0)+...
         Ir_31.*t17.*t140.*(3.0./8.0)-Ir_31.*t17.*t142.*(3.0./8.0)-Ir_22.*t4.*t174.*(1.0./8.0)+Ir_22.*t4.*t175.*(1.0./8.0)-Ir_11.*t17.*t174.*(1.0./8.0)+...
         Ir_11.*t4.*t188.*(1.0./1.6e1)+Ir_11.*t17.*t175.*(1.0./8.0)+Ir_11.*t4.*t189.*(1.0./3.2e1)-Ir_11.*t17.*t176.*(3.0./8.0)-Ir_11.*t4.*t190.*(1.0./3.2e1)-...
         Ir_11.*t17.*t177.*(3.0./1.6e1)+Ir_11.*t17.*t178.*(3.0./1.6e1)+Ir_33.*t4.*t174.*(1.0./8.0)-Ir_32.*t4.*t176.*(1.0./8.0)-Ir_33.*t4.*t175.*(1.0./8.0)-...
         Ir_32.*t4.*t177.*(1.0./8.0)-Ir_32.*t4.*t178.*(1.0./8.0)+Ir_32.*t17.*t174.*(1.0./2.0)+Ir_32.*t17.*t175.*(1.0./2.0)+Ir_33.*t17.*t174.*(1.0./8.0)-...
         Ir_33.*t4.*t188.*(1.0./1.6e1)-Ir_33.*t17.*t175.*(1.0./8.0)-Ir_33.*t4.*t189.*(1.0./3.2e1)+Ir_33.*t17.*t176.*(3.0./8.0)+Ir_33.*t4.*t190.*(1.0./3.2e1)+...
         Ir_33.*t17.*t177.*(3.0./1.6e1)-Ir_33.*t17.*t178.*(3.0./1.6e1)+Ir_31.*t4.*t202.*(1.0./8.0)-Ir_31.*t4.*t220.*(1.0./8.0)-Ir_31.*t4.*t221.*(1.0./1.6e1)+...
         Ir_31.*t4.*t222.*(1.0./1.6e1)-Ii_21.*t5.*cos(phi_i.*-3.0+t19+t20).*(1.0./8.0)+Ii_31.*t5.*cos(phi_i.*-2.0+t19+t20).*(1.0./8.0)-Ii_31.*t5.*cos(phi_i.*-4.0+...
         t19+t20).*(1.0./1.6e1)-Io_21.*t8.*cos(phi_o.*-3.0+t19+t24).*(1.0./8.0)+Io_31.*t8.*cos(phi_o.*-2.0+t19+t24).*(1.0./8.0)-Io_31.*t8.*cos(phi_o.*-4.0+t19+...
         t24).*(1.0./1.6e1)+Il_21.*t15.*cos(t55).*(1.0./2.0)+Il_21.*t15.*cos(t167).*(1.0./2.0)+Ir_21.*t17.*cos(t61).*(1.0./2.0)+Ir_21.*t17.*cos(t173).*(1.0./2.0)-...
         Ii_21.*phip_i.*t73.*thetap.*(1.0./8.0)-Ii_21.*phip_i.*t81.*thetap.*(3.0./8.0)-Ii_32.*phip_i.*t70.*thetap.*(1.0./4.0)-Ii_31.*phip_i.*t76.*thetap.*(1.0./4.0)-...
         Ii_31.*phip_i.*t78.*thetap.*(1.0./4.0)-Ii_11.*phip_i.*t99.*thetap.*(1.0./8.0)-Ii_22.*phip_i.*t95.*thetap.*(1.0./4.0)-Ii_33.*phip_i.*t96.*thetap.*(1.0./4.0)-...
         Ii_33.*phip_i.*t98.*thetap.*(1.0./8.0)-Ii_32.*phip_i.*t113.*thetap.*(3.0./8.0)-Ii_32.*phip_i.*t114.*thetap.*(3.0./8.0)-Ii_21.*phip_i.*t144.*thetap.*(1.0./4.0)-...
         Ii_11.*phip_i.*t158.*thetap.*(1.0./2.0)-Ii_21.*phip_i.*t148.*thetap.*(3.0./4.0)-Ii_33.*phip_i.*t157.*thetap.*(1.0./2.0)-Ii_11.*phip_i.*t206.*thetap.*(3.0./4.0)-...
         Ii_32.*phip_i.*t191.*thetap.*(1.0./4.0)-Ii_32.*phip_i.*t192.*thetap.*(3.0./4.0)-Ii_32.*phip_i.*t193.*thetap.*(3.0./4.0)-Ii_22.*phip_i.*t205.*thetap.*(1.0./2.0)+...
         Il_21.*phip_l.*t12.*thetap.*(1.0./4.0)-Il_32.*phip_l.*t16.*thetap.*(1.0./4.0)-Il_21.*phip_l.*t31.*thetap.*(1.0./8.0)+Il_21.*phip_l.*t33.*thetap.*(1.0./8.0)-...
         Il_21.*phip_l.*t39.*thetap.*(1.0./4.0)-Il_21.*phip_l.*t42.*thetap.*(3.0./4.0)-Il_11.*phip_l.*t66.*thetap.*(1.0./2.0)-Il_32.*phip_l.*t52.*thetap.*(3.0./8.0)+...
         Il_32.*phip_l.*t53.*thetap.*(3.0./8.0)+Il_32.*phip_l.*t56.*thetap.*(1.0./4.0)-Il_32.*phip_l.*t57.*thetap.*(3.0./4.0)+Il_33.*phip_l.*t66.*thetap.*(1.0./2.0)+...
         Il_21.*phip_l.*t132.*thetap.*(3.0./4.0)+Il_21.*phip_l.*t134.*thetap.*(3.0./8.0)-Il_31.*phip_l.*t124.*thetap.*(1.0./4.0)-Il_21.*phip_l.*t136.*thetap.*(3.0./8.0)-...
         Il_31.*phip_l.*t126.*thetap.*(1.0./4.0)+Il_22.*phip_l.*t168.*thetap.*(1.0./4.0)+Il_22.*phip_l.*t169.*thetap.*(1.0./4.0)-Il_11.*phip_l.*t182.*thetap.*(1.0./2.0)-...
         Il_11.*phip_l.*t183.*thetap.*(1.0./8.0)-Il_11.*phip_l.*t184.*thetap.*(1.0./8.0)-Il_33.*phip_l.*t168.*thetap.*(1.0./4.0)+Il_32.*phip_l.*t170.*thetap.*(3.0./4.0)-...
         Il_33.*phip_l.*t169.*thetap.*(1.0./4.0)+Il_32.*phip_l.*t171.*thetap.*(3.0./8.0)-Il_32.*phip_l.*t172.*thetap.*(3.0./8.0)+Il_33.*phip_l.*t182.*thetap.*(1.0./2.0)+...
         Il_33.*phip_l.*t183.*thetap.*(1.0./8.0)+Il_33.*phip_l.*t184.*thetap.*(1.0./8.0)-Il_11.*phip_l.*t214.*thetap.*(3.0./4.0)+Il_31.*phip_l.*t201.*thetap-...
         Il_22.*phip_l.*t213.*thetap.*(1.0./2.0)+Il_33.*phip_l.*t213.*thetap.*(1.0./2.0)+Il_33.*phip_l.*t214.*thetap.*(3.0./4.0)+Il_31.*phip_l.*t217.*thetap+...
         Il_31.*phip_l.*t218.*thetap.*(1.0./4.0)+Il_31.*phip_l.*t219.*thetap.*(1.0./4.0)-Io_32.*phip_o.*t71.*thetap.*(1.0./4.0)-Io_21.*phip_o.*t83.*thetap.*(1.0./8.0)-...
         Io_21.*phip_o.*t91.*thetap.*(3.0./8.0)-Io_31.*phip_o.*t86.*thetap.*(1.0./4.0)-Io_11.*phip_o.*t107.*thetap.*(1.0./8.0)-Io_31.*phip_o.*t88.*thetap.*(1.0./4.0)-...
         Io_22.*phip_o.*t103.*thetap.*(1.0./4.0)-Io_33.*phip_o.*t104.*thetap.*(1.0./4.0)-Io_33.*phip_o.*t106.*thetap.*(1.0./8.0)-Io_32.*phip_o.*t116.*thetap.*(3.0./8.0)-...
         Io_32.*phip_o.*t117.*thetap.*(3.0./8.0)-Io_21.*phip_o.*t150.*thetap.*(1.0./4.0)-Io_11.*phip_o.*t162.*thetap.*(1.0./2.0)-Io_21.*phip_o.*t154.*thetap.*(3.0./4.0)-...
         Io_33.*phip_o.*t161.*thetap.*(1.0./2.0)-Io_11.*phip_o.*t208.*thetap.*(3.0./4.0)-Io_32.*phip_o.*t196.*thetap.*(1.0./4.0)-Io_22.*phip_o.*t207.*thetap.*(1.0./2.0)-...
         Io_32.*phip_o.*t197.*thetap.*(3.0./4.0)-Io_32.*phip_o.*t198.*thetap.*(3.0./4.0)+Ir_21.*phip_r.*t14.*thetap.*(1.0./4.0)-Ir_32.*phip_r.*t18.*thetap.*(1.0./4.0)-...
         Ir_21.*phip_r.*t35.*thetap.*(1.0./8.0)+Ir_21.*phip_r.*t37.*thetap.*(1.0./8.0)-Ir_21.*phip_r.*t44.*thetap.*(1.0./4.0)-Ir_21.*phip_r.*t47.*thetap.*(3.0./4.0)-...
         Ir_11.*phip_r.*t69.*thetap.*(1.0./2.0)-Ir_32.*phip_r.*t58.*thetap.*(3.0./8.0)+Ir_32.*phip_r.*t59.*thetap.*(3.0./8.0)+Ir_32.*phip_r.*t62.*thetap.*(1.0./4.0)-...
         Ir_32.*phip_r.*t63.*thetap.*(3.0./4.0)+Ir_33.*phip_r.*t69.*thetap.*(1.0./2.0)+Ir_21.*phip_r.*t138.*thetap.*(3.0./4.0)-Ir_31.*phip_r.*t128.*thetap.*(1.0./4.0)+...
         Ir_21.*phip_r.*t140.*thetap.*(3.0./8.0)-Ir_31.*phip_r.*t130.*thetap.*(1.0./4.0)-Ir_21.*phip_r.*t142.*thetap.*(3.0./8.0)+Ir_22.*phip_r.*t174.*thetap.*(1.0./4.0)+...
         Ir_22.*phip_r.*t175.*thetap.*(1.0./4.0)-Ir_11.*phip_r.*t188.*thetap.*(1.0./2.0)-Ir_11.*phip_r.*t189.*thetap.*(1.0./8.0)-Ir_11.*phip_r.*t190.*thetap.*(1.0./8.0)-...
         Ir_33.*phip_r.*t174.*thetap.*(1.0./4.0)+Ir_32.*phip_r.*t176.*thetap.*(3.0./4.0)-Ir_33.*phip_r.*t175.*thetap.*(1.0./4.0)+Ir_32.*phip_r.*t177.*thetap.*(3.0./8.0)-...
         Ir_32.*phip_r.*t178.*thetap.*(3.0./8.0)+Ir_33.*phip_r.*t188.*thetap.*(1.0./2.0)+Ir_33.*phip_r.*t189.*thetap.*(1.0./8.0)+Ir_33.*phip_r.*t190.*thetap.*(1.0./8.0)-...
         Ir_11.*phip_r.*t216.*thetap.*(3.0./4.0)+Ir_31.*phip_r.*t202.*thetap-Ir_22.*phip_r.*t215.*thetap.*(1.0./2.0)+Ir_33.*phip_r.*t215.*thetap.*(1.0./2.0)+...
         Ir_33.*phip_r.*t216.*thetap.*(3.0./4.0)+Ir_31.*phip_r.*t220.*thetap+Ir_31.*phip_r.*t221.*thetap.*(1.0./4.0)+Ir_31.*phip_r.*t222.*thetap.*(1.0./4.0)+...
         Il_31.*phip_l.*thetap.*cos(t54).*(1.0./2.0)+Il_31.*phip_l.*thetap.*cos(t64).*(3.0./2.0)+Ir_31.*phip_r.*thetap.*cos(t60).*(1.0./2.0)+Ir_31.*phip_r.*thetap.*cos(t67).*(3.0./2.0)-...
         Ii_21.*deltap_i.*phip_i.*t73.*(1.0./8.0)-Ii_21.*deltap_i.*phip_i.*t81.*(3.0./8.0)-Ii_32.*deltap_i.*phip_i.*t70.*(1.0./4.0)-Ii_31.*deltap_i.*phip_i.*t76.*(1.0./4.0)-...
         Ii_31.*deltap_i.*phip_i.*t78.*(1.0./4.0)-Ii_11.*deltap_i.*phip_i.*t99.*(1.0./8.0)-Ii_22.*deltap_i.*phip_i.*t95.*(1.0./4.0)-Ii_33.*deltap_i.*phip_i.*t96.*(1.0./4.0)-...
         Ii_33.*deltap_i.*phip_i.*t98.*(1.0./8.0)-Ii_32.*deltap_i.*phip_i.*t113.*(3.0./8.0)-Ii_32.*deltap_i.*phip_i.*t114.*(3.0./8.0)-Ii_21.*deltap_i.*phip_i.*t144.*(1.0./4.0)-...
         Ii_11.*deltap_i.*phip_i.*t158.*(1.0./2.0)-Ii_21.*deltap_i.*phip_i.*t148.*(3.0./4.0)-Ii_33.*deltap_i.*phip_i.*t157.*(1.0./2.0)-Ii_11.*deltap_i.*phip_i.*t206.*(3.0./4.0)-...
         Ii_32.*deltap_i.*phip_i.*t191.*(1.0./4.0)-Ii_32.*deltap_i.*phip_i.*t192.*(3.0./4.0)-Ii_32.*deltap_i.*phip_i.*t193.*(3.0./4.0)-Ii_22.*deltap_i.*phip_i.*t205.*(1.0./2.0)-...
         Io_32.*deltap_o.*phip_o.*t71.*(1.0./4.0)-Io_21.*deltap_o.*phip_o.*t83.*(1.0./8.0)-Io_21.*deltap_o.*phip_o.*t91.*(3.0./8.0)-Io_31.*deltap_o.*phip_o.*t86.*(1.0./4.0)-...
         Io_11.*deltap_o.*phip_o.*t107.*(1.0./8.0)-Io_31.*deltap_o.*phip_o.*t88.*(1.0./4.0)-Io_22.*deltap_o.*phip_o.*t103.*(1.0./4.0)-Io_33.*deltap_o.*phip_o.*t104.*(1.0./4.0)-...
         Io_33.*deltap_o.*phip_o.*t106.*(1.0./8.0)-Io_32.*deltap_o.*phip_o.*t116.*(3.0./8.0)-Io_32.*deltap_o.*phip_o.*t117.*(3.0./8.0)-Io_21.*deltap_o.*phip_o.*t150.*(1.0./4.0)-...
         Io_11.*deltap_o.*phip_o.*t162.*(1.0./2.0)-Io_21.*deltap_o.*phip_o.*t154.*(3.0./4.0)-Io_33.*deltap_o.*phip_o.*t161.*(1.0./2.0)-Io_11.*deltap_o.*phip_o.*t208.*(3.0./4.0)-...
         Io_32.*deltap_o.*phip_o.*t196.*(1.0./4.0)-Io_22.*deltap_o.*phip_o.*t207.*(1.0./2.0)-Io_32.*deltap_o.*phip_o.*t197.*(3.0./4.0)-Io_32.*deltap_o.*phip_o.*t198.*(3.0./4.0)-...
         Ii_33.*deltap_i.*t7.*thetap.*(1.0./4.0)-Ii_21.*deltap_i.*t81.*thetap.*(1.0./4.0)-Ii_32.*deltap_i.*t70.*thetap.*(1.0./4.0)-Ii_31.*deltap_i.*t76.*thetap.*(1.0./4.0)-...
         Ii_11.*deltap_i.*t98.*thetap.*(1.0./1.6e1)-Ii_11.*deltap_i.*t99.*thetap.*(1.0./1.6e1)-Ii_33.*deltap_i.*t95.*thetap.*(1.0./4.0)-Ii_21.*deltap_i.*t108.*thetap.*(1.0./4.0)-...
         Ii_33.*deltap_i.*t96.*thetap.*(1.0./4.0)-Ii_22.*deltap_i.*t120.*thetap.*(1.0./2.0)-Ii_32.*deltap_i.*t112.*thetap.*(3.0./4.0)-Ii_32.*deltap_i.*t114.*thetap.*(1.0./4.0)-...
         Ii_21.*deltap_i.*t146.*thetap.*(1.0./4.0)-Ii_11.*deltap_i.*t157.*thetap.*(1.0./8.0)-Ii_11.*deltap_i.*t158.*thetap.*(1.0./8.0)-Ii_21.*deltap_i.*t148.*thetap.*(1.0./4.0)-...
         Ii_31.*deltap_i.*t163.*thetap.*(1.0./4.0)-Ii_32.*deltap_i.*t193.*thetap.*(1.0./4.0)-Ii_31.*deltap_i.*t203.*thetap.*(1.0./8.0)-Io_33.*deltap_o.*t10.*thetap.*(1.0./4.0)-...
         Io_32.*deltap_o.*t71.*thetap.*(1.0./4.0)-Io_21.*deltap_o.*t91.*thetap.*(1.0./4.0)-Io_11.*deltap_o.*t106.*thetap.*(1.0./1.6e1)-Io_31.*deltap_o.*t86.*thetap.*(1.0./4.0)-...
         Io_11.*deltap_o.*t107.*thetap.*(1.0./1.6e1)-Io_21.*deltap_o.*t110.*thetap.*(1.0./4.0)-Io_33.*deltap_o.*t103.*thetap.*(1.0./4.0)-Io_33.*deltap_o.*t104.*thetap.*(1.0./4.0)-...
         Io_22.*deltap_o.*t122.*thetap.*(1.0./2.0)-Io_32.*deltap_o.*t115.*thetap.*(3.0./4.0)-Io_32.*deltap_o.*t117.*thetap.*(1.0./4.0)-Io_11.*deltap_o.*t161.*thetap.*(1.0./8.0)-...
         Io_11.*deltap_o.*t162.*thetap.*(1.0./8.0)-Io_21.*deltap_o.*t152.*thetap.*(1.0./4.0)-Io_21.*deltap_o.*t154.*thetap.*(1.0./4.0)-Io_31.*deltap_o.*t165.*thetap.*(1.0./4.0)-...
         Io_32.*deltap_o.*t198.*thetap.*(1.0./4.0)-Io_31.*deltap_o.*t204.*thetap.*(1.0./8.0);
    
    Q41 = aux3-Ii_33.*t4.*t7.*(1.0./8.0)-Ii_33.*t5.*t7.*(1.0./8.0)-Ii_22.*t23.*t28.*(1.0./4.0)-Ii_31.*t23.*t49.*(1.0./4.0)-Ii_21.*t4.*t81.*(1.0./8.0)-Ii_32.*t4.*t70.*(1.0./8.0)-...
         Ii_21.*t5.*t81.*(1.0./8.0)-Ii_32.*t5.*t70.*(1.0./8.0)-Ii_31.*t4.*t76.*(1.0./8.0)-Ii_31.*t5.*t76.*(1.0./8.0)-Ii_11.*t4.*t98.*(1.0./3.2e1)-Ii_11.*t4.*t99.*(1.0./3.2e1)-...
         Ii_11.*t5.*t98.*(1.0./3.2e1)+Ii_31.*t5.*t78.*(1.0./8.0)-Ii_11.*t5.*t99.*(1.0./3.2e1)-Ii_33.*t23.*t70.*(1.0./8.0)-Ii_31.*t23.*t73.*(1.0./8.0)-Ii_31.*t23.*t76.*(1.0./4.0)-...
         Ii_33.*t4.*t95.*(1.0./8.0)-Ii_21.*t4.*t108.*(1.0./8.0)-Ii_33.*t4.*t96.*(1.0./8.0)-Ii_33.*t5.*t95.*(1.0./8.0)-Ii_21.*t5.*t108.*(1.0./8.0)-Ii_33.*t5.*t96.*(1.0./8.0)-...
         Ii_31.*t23.*t81.*(3.0./8.0)-Ii_22.*t4.*t120.*(1.0./4.0)-Ii_22.*t5.*t120.*(1.0./4.0)-Ii_32.*t4.*t112.*(3.0./8.0)-Ii_32.*t5.*t112.*(3.0./8.0)-Ii_32.*t4.*t114.*(1.0./8.0)-...
         Ii_32.*t23.*t95.*(1.0./2.0)-Ii_32.*t5.*t114.*(1.0./8.0)-Ii_33.*t23.*t95.*(1.0./8.0)-Ii_33.*t23.*t96.*(1.0./8.0)-Ii_22.*t23.*t112.*(1.0./4.0)-Ii_22.*t23.*t120.*(1.0./2.0)-...
         Ii_32.*t23.*t112.*(1.0./2.0)-Ii_33.*t23.*t113.*(3.0./1.6e1)-Ii_33.*t23.*t114.*(3.0./1.6e1)-Ii_21.*t4.*t146.*(1.0./8.0)-Ii_11.*t4.*t157.*(1.0./1.6e1)-Ii_21.*t5.*t146.*(1.0./8.0)-...
         Ii_11.*t4.*t158.*(1.0./1.6e1)-Ii_11.*t5.*t157.*(1.0./1.6e1)-Ii_21.*t4.*t148.*(1.0./8.0)-Ii_11.*t5.*t158.*(1.0./1.6e1)-Ii_21.*t5.*t148.*(1.0./8.0)-Ii_31.*t4.*t163.*(1.0./8.0)-...
         Ii_31.*t5.*t163.*(1.0./8.0)-Ii_31.*t23.*t148.*(3.0./4.0)-Ii_32.*t4.*t193.*(1.0./8.0)-Ii_32.*t5.*t193.*(1.0./8.0)-Ii_31.*t4.*t203.*(1.0./1.6e1)-Ii_31.*t5.*t203.*(1.0./1.6e1)-...
         Ii_33.*t23.*t191.*(1.0./8.0)-Ii_33.*t23.*t192.*(3.0./8.0)-Ii_33.*t23.*t193.*(3.0./8.0)-Ii_32.*t23.*t287.*(1.0./2.0)-Ii_21.*phip_i.*t73.*thetap.*(1.0./8.0)-...
         Ii_21.*phip_i.*t81.*thetap.*(3.0./8.0)-Ii_32.*phip_i.*t70.*thetap.*(1.0./4.0)-Ii_31.*phip_i.*t76.*thetap.*(1.0./4.0)-Ii_31.*phip_i.*t78.*thetap.*(1.0./4.0)-...
         Ii_11.*phip_i.*t99.*thetap.*(1.0./8.0)-Ii_22.*phip_i.*t95.*thetap.*(1.0./4.0)-Ii_33.*phip_i.*t96.*thetap.*(1.0./4.0)-Ii_33.*phip_i.*t98.*thetap.*(1.0./8.0)-...
         Ii_32.*phip_i.*t113.*thetap.*(3.0./8.0)-Ii_32.*phip_i.*t114.*thetap.*(3.0./8.0)-Ii_21.*phip_i.*t144.*thetap.*(1.0./4.0)-Ii_11.*phip_i.*t158.*thetap.*(1.0./2.0)-...
         Ii_21.*phip_i.*t148.*thetap.*(3.0./4.0)-Ii_33.*phip_i.*t157.*thetap.*(1.0./2.0)-Ii_11.*phip_i.*t206.*thetap.*(3.0./4.0)-Ii_32.*phip_i.*t191.*thetap.*(1.0./4.0)-...
         Ii_32.*phip_i.*t192.*thetap.*(3.0./4.0)-Ii_32.*phip_i.*t193.*thetap.*(3.0./4.0)-Ii_22.*phip_i.*t205.*thetap.*(1.0./2.0)-Ii_21.*deltap_i.*phip_i.*t73.*(1.0./8.0)-...
         Ii_21.*deltap_i.*phip_i.*t81.*(3.0./8.0)-Ii_32.*deltap_i.*phip_i.*t70.*(1.0./4.0)-Ii_31.*deltap_i.*phip_i.*t76.*(1.0./4.0)-Ii_31.*deltap_i.*phip_i.*t78.*(1.0./4.0)-...
         Ii_11.*deltap_i.*phip_i.*t99.*(1.0./8.0)-Ii_22.*deltap_i.*phip_i.*t95.*(1.0./4.0)-Ii_33.*deltap_i.*phip_i.*t96.*(1.0./4.0)-Ii_33.*deltap_i.*phip_i.*t98.*(1.0./8.0)-...
         Ii_32.*deltap_i.*phip_i.*t113.*(3.0./8.0)-Ii_32.*deltap_i.*phip_i.*t114.*(3.0./8.0)-Ii_21.*deltap_i.*phip_i.*t144.*(1.0./4.0)-Ii_11.*deltap_i.*phip_i.*t158.*(1.0./2.0)-...
         Ii_21.*deltap_i.*phip_i.*t148.*(3.0./4.0)-Ii_33.*deltap_i.*phip_i.*t157.*(1.0./2.0)-Ii_11.*deltap_i.*phip_i.*t206.*(3.0./4.0)-Ii_32.*deltap_i.*phip_i.*t191.*(1.0./4.0)-...
         Ii_32.*deltap_i.*phip_i.*t192.*(3.0./4.0)-Ii_32.*deltap_i.*phip_i.*t193.*(3.0./4.0)-Ii_22.*deltap_i.*phip_i.*t205.*(1.0./2.0)-Ii_33.*deltap_i.*t7.*thetap.*(1.0./4.0)-...
         Ii_21.*deltap_i.*t81.*thetap.*(1.0./4.0)-Ii_32.*deltap_i.*t70.*thetap.*(1.0./4.0)-Ii_31.*deltap_i.*t76.*thetap.*(1.0./4.0)-Ii_11.*deltap_i.*t98.*thetap.*(1.0./1.6e1)-...
         Ii_11.*deltap_i.*t99.*thetap.*(1.0./1.6e1)-Ii_33.*deltap_i.*t95.*thetap.*(1.0./4.0)-Ii_21.*deltap_i.*t108.*thetap.*(1.0./4.0)-Ii_33.*deltap_i.*t96.*thetap.*(1.0./4.0)-...
         Ii_22.*deltap_i.*t120.*thetap.*(1.0./2.0)-Ii_32.*deltap_i.*t112.*thetap.*(3.0./4.0)-Ii_32.*deltap_i.*t114.*thetap.*(1.0./4.0)-Ii_21.*deltap_i.*t146.*thetap.*(1.0./4.0)-...
         Ii_11.*deltap_i.*t157.*thetap.*(1.0./8.0)-Ii_11.*deltap_i.*t158.*thetap.*(1.0./8.0)-Ii_21.*deltap_i.*t148.*thetap.*(1.0./4.0)-Ii_31.*deltap_i.*t163.*thetap.*(1.0./4.0)-...
         Ii_32.*deltap_i.*t193.*thetap.*(1.0./4.0)-Ii_31.*deltap_i.*t203.*thetap.*(1.0./8.0);
     
    Q51 = aux2-Io_33.*t4.*t10.*(1.0./8.0)-Io_33.*t8.*t10.*(1.0./8.0)-...
            Io_22.*t27.*t29.*(1.0./4.0)-Io_32.*t4.*t71.*(1.0./8.0)-Io_31.*t27.*t51.*(1.0./4.0)-Io_32.*t8.*t71.*(1.0./8.0)-Io_21.*t4.*t91.*(1.0./8.0)-Io_21.*t8.*t91.*(1.0./8.0)-...
            Io_11.*t4.*t106.*(1.0./3.2e1)-Io_31.*t4.*t86.*(1.0./8.0)-Io_11.*t4.*t107.*(1.0./3.2e1)-Io_11.*t8.*t106.*(1.0./3.2e1)-Io_31.*t8.*t86.*(1.0./8.0)-Io_11.*t8.*t107.*(1.0./3.2e1)+...
            Io_31.*t8.*t88.*(1.0./8.0)-Io_33.*t27.*t71.*(1.0./8.0)-Io_21.*t4.*t110.*(1.0./8.0)-Io_21.*t8.*t110.*(1.0./8.0)-Io_33.*t4.*t103.*(1.0./8.0)-Io_31.*t27.*t83.*(1.0./8.0)-...
            Io_33.*t4.*t104.*(1.0./8.0)-Io_31.*t27.*t86.*(1.0./4.0)-Io_33.*t8.*t103.*(1.0./8.0)-Io_33.*t8.*t104.*(1.0./8.0)-Io_22.*t4.*t122.*(1.0./4.0)-Io_31.*t27.*t91.*(3.0./8.0)-...
            Io_32.*t4.*t115.*(3.0./8.0)-Io_22.*t8.*t122.*(1.0./4.0)-Io_32.*t4.*t117.*(1.0./8.0)-Io_32.*t8.*t115.*(3.0./8.0)-Io_32.*t8.*t117.*(1.0./8.0)-Io_32.*t27.*t103.*(1.0./2.0)-...
            Io_33.*t27.*t103.*(1.0./8.0)-Io_22.*t27.*t115.*(1.0./4.0)-Io_33.*t27.*t104.*(1.0./8.0)-Io_22.*t27.*t122.*(1.0./2.0)-Io_32.*t27.*t115.*(1.0./2.0)-Io_11.*t4.*t161.*(1.0./1.6e1)-...
            Io_33.*t27.*t116.*(3.0./1.6e1)-Io_11.*t4.*t162.*(1.0./1.6e1)-Io_21.*t4.*t152.*(1.0./8.0)-Io_33.*t27.*t117.*(3.0./1.6e1)-Io_21.*t4.*t154.*(1.0./8.0)-Io_11.*t8.*t161.*(1.0./1.6e1)-...
            Io_11.*t8.*t162.*(1.0./1.6e1)-Io_21.*t8.*t152.*(1.0./8.0)-Io_21.*t8.*t154.*(1.0./8.0)-Io_31.*t4.*t165.*(1.0./8.0)-Io_31.*t8.*t165.*(1.0./8.0)-Io_31.*t27.*t154.*(3.0./4.0)-...
            Io_32.*t4.*t198.*(1.0./8.0)-Io_32.*t8.*t198.*(1.0./8.0)-Io_31.*t4.*t204.*(1.0./1.6e1)-Io_31.*t8.*t204.*(1.0./1.6e1)-Io_33.*t27.*t196.*(1.0./8.0)-Io_33.*t27.*t197.*(3.0./8.0)-...
            Io_33.*t27.*t198.*(3.0./8.0)-Io_32.*t27.*t418.*(1.0./2.0)-Io_32.*phip_o.*t71.*thetap.*(1.0./4.0)-Io_21.*phip_o.*t83.*thetap.*(1.0./8.0)-Io_21.*phip_o.*t91.*thetap.*(3.0./8.0)-...
            Io_31.*phip_o.*t86.*thetap.*(1.0./4.0)-Io_11.*phip_o.*t107.*thetap.*(1.0./8.0)-Io_31.*phip_o.*t88.*thetap.*(1.0./4.0)-...
            Io_22.*phip_o.*t103.*thetap.*(1.0./4.0)-Io_33.*phip_o.*t104.*thetap.*(1.0./4.0)-...
            Io_33.*phip_o.*t106.*thetap.*(1.0./8.0)-Io_32.*phip_o.*t116.*thetap.*(3.0./8.0)-Io_32.*phip_o.*t117.*thetap.*(3.0./8.0)-...
            Io_21.*phip_o.*t150.*thetap.*(1.0./4.0)-Io_11.*phip_o.*t162.*thetap.*(1.0./2.0)-...
            Io_21.*phip_o.*t154.*thetap.*(3.0./4.0)-Io_33.*phip_o.*t161.*thetap.*(1.0./2.0)-Io_11.*phip_o.*t208.*thetap.*(3.0./4.0)-...
            Io_32.*phip_o.*t196.*thetap.*(1.0./4.0)-Io_22.*phip_o.*t207.*thetap.*(1.0./2.0)-...
            Io_32.*phip_o.*t197.*thetap.*(3.0./4.0)-Io_32.*phip_o.*t198.*thetap.*(3.0./4.0)-Io_32.*deltap_o.*phip_o.*t71.*(1.0./4.0)-...
            Io_21.*deltap_o.*phip_o.*t83.*(1.0./8.0)-Io_21.*deltap_o.*phip_o.*t91.*(3.0./8.0)-...
            Io_31.*deltap_o.*phip_o.*t86.*(1.0./4.0)-Io_11.*deltap_o.*phip_o.*t107.*(1.0./8.0)-Io_31.*deltap_o.*phip_o.*t88.*(1.0./4.0)-...
            Io_22.*deltap_o.*phip_o.*t103.*(1.0./4.0)-Io_33.*deltap_o.*phip_o.*t104.*(1.0./4.0)-...
            Io_33.*deltap_o.*phip_o.*t106.*(1.0./8.0)-Io_32.*deltap_o.*phip_o.*t116.*(3.0./8.0)-Io_32.*deltap_o.*phip_o.*t117.*(3.0./8.0)-...
            Io_21.*deltap_o.*phip_o.*t150.*(1.0./4.0)-Io_11.*deltap_o.*phip_o.*t162.*(1.0./2.0)-...
            Io_21.*deltap_o.*phip_o.*t154.*(3.0./4.0)-Io_33.*deltap_o.*phip_o.*t161.*(1.0./2.0)-Io_11.*deltap_o.*phip_o.*t208.*(3.0./4.0)-...
            Io_32.*deltap_o.*phip_o.*t196.*(1.0./4.0)-Io_22.*deltap_o.*phip_o.*t207.*(1.0./2.0)-...
            Io_32.*deltap_o.*phip_o.*t197.*(3.0./4.0)-Io_32.*deltap_o.*phip_o.*t198.*(3.0./4.0)-Io_33.*deltap_o.*t10.*thetap.*(1.0./4.0)-...
            Io_32.*deltap_o.*t71.*thetap.*(1.0./4.0)-Io_21.*deltap_o.*t91.*thetap.*(1.0./4.0)-...
            Io_11.*deltap_o.*t106.*thetap.*(1.0./1.6e1)-Io_31.*deltap_o.*t86.*thetap.*(1.0./4.0)-Io_11.*deltap_o.*t107.*thetap.*(1.0./1.6e1)-...
            Io_21.*deltap_o.*t110.*thetap.*(1.0./4.0)-Io_33.*deltap_o.*t103.*thetap.*(1.0./4.0)-...
            Io_33.*deltap_o.*t104.*thetap.*(1.0./4.0)-Io_22.*deltap_o.*t122.*thetap.*(1.0./2.0)-Io_32.*deltap_o.*t115.*thetap.*(3.0./4.0)-...
            Io_32.*deltap_o.*t117.*thetap.*(1.0./4.0)-Io_11.*deltap_o.*t161.*thetap.*(1.0./8.0)-...
            Io_11.*deltap_o.*t162.*thetap.*(1.0./8.0)-Io_21.*deltap_o.*t152.*thetap.*(1.0./4.0)-Io_21.*deltap_o.*t154.*thetap.*(1.0./4.0)-...
            Io_31.*deltap_o.*t165.*thetap.*(1.0./4.0)-Io_32.*deltap_o.*t198.*thetap.*(1.0./4.0)-Io_31.*deltap_o.*t204.*thetap.*(1.0./8.0);
     
    Q61 = f_phi_i+Ii_11.*t4.*t206.*(3.0./8.0)+Ii_11.*t5.*t206.*(3.0./8.0)+Ii_22.*t4.*t205.*(1.0./4.0)+Ii_22.*t5.*t205.*(1.0./4.0)+Ii_11.*t23.*t205.*(1.0./4.0)-...
         Ii_33.*t4.*t205.*(1.0./4.0)-Ii_33.*t4.*t206.*(3.0./8.0)-...
         Ii_33.*t5.*t205.*(1.0./4.0)-Ii_31.*t4.*t209.*(1.0./4.0)-Ii_33.*t5.*t206.*(3.0./8.0)-Ii_31.*t4.*t210.*(3.0./4.0)-Ii_31.*t5.*t209.*(1.0./4.0)-...
         Ii_31.*t5.*t210.*(3.0./4.0)-Ii_33.*t23.*t205.*(1.0./4.0)...
         -Ii_31.*t23.*t209.*(1.0./2.0)+Ii_32.*t2.*t4.*t485.*(1.0./2.0)+Ii_32.*t2.*t5.*t485.*(1.0./2.0)+Ii_32.*t3.*t4.*t486.*(1.0./2.0)+Ii_32.*t3.*t5.*t486.*(1.0./2.0)-...
         Ii_32.*t4.*t118.*t487-Ii_32.*t5.*t118.*t487-Ii_32.*t4.*t488.*t489-...
         Ii_32.*t5.*t488.*t489+Ii_11.*deltap_i.*t206.*thetap.*(3.0./4.0)+Ii_22.*deltap_i.*t205.*thetap.*(1.0./2.0)-Ii_33.*deltap_i.*t205.*thetap.*(1.0./2.0)-...
         Ii_33.*deltap_i.*t206.*thetap.*(3.0./4.0)-Ii_31.*deltap_i.*t209.*thetap.*(1.0./2.0)-...
         Ii_31.*deltap_i.*t210.*thetap.*(3.0./2.0)-Ii_11.*deltap_i.*phip_i.*t118.*t487.*(1.0./2.0)+Ii_22.*deltap_i.*phip_i.*t118.*t487-...
         Ii_33.*deltap_i.*phip_i.*t118.*t487.*(1.0./2.0)-Ii_11.*deltap_i.*phip_i.*t488.*t489.*(1.0./2.0)+Ii_22.*deltap_i.*phip_i.*t488.*t489-...
         Ii_33.*deltap_i.*phip_i.*t488.*t489.*(1.0./2.0)+Ii_32.*deltap_i.*t2.*t485.*thetap+Ii_32.*deltap_i.*t3.*t486.*thetap-...
         Ii_32.*deltap_i.*t118.*t487.*thetap.*2.0-Ii_32.*deltap_i.*t488.*t489.*thetap.*2.0-Ii_11.*phip_i.*t118.*t487.*thetap.*(1.0./2.0)+Ii_22.*phip_i.*t118.*t487.*thetap-...
         Ii_33.*phip_i.*t118.*t487.*thetap.*(1.0./2.0)-Ii_11.*phip_i.*t488.*t489.*thetap.*(1.0./2.0)+Ii_22.*phip_i.*t488.*t489.*thetap-...
         Ii_33.*phip_i.*t488.*t489.*thetap.*(1.0./2.0)-Ii_11.*t2.*t4.*t206.*t486.*(1.0./2.0)+Ii_11.*t3.*t4.*t206.*t485.*(1.0./2.0)-Ii_11.*t2.*t5.*t206.*t486.*(1.0./2.0)+...
         Ii_11.*t3.*t5.*t206.*t485.*(1.0./2.0)-Ii_21.*t2.*t4.*t205.*t485.*(1.0./2.0)-Ii_21.*t2.*t5.*t205.*t485.*(1.0./2.0)-Ii_21.*t3.*t4.*t205.*t486.*(1.0./2.0)-...
         Ii_21.*t3.*t5.*t205.*t486.*(1.0./2.0)+Ii_33.*t2.*t4.*t206.*t486.*(1.0./2.0)-Ii_33.*t3.*t4.*t206.*t485.*(1.0./2.0)+Ii_32.*t2.*t4.*t209.*t485.*(1.0./2.0)+...
         Ii_33.*t2.*t5.*t206.*t486.*(1.0./2.0)-Ii_33.*t3.*t5.*t206.*t485.*(1.0./2.0)+Ii_31.*t2.*t4.*t210.*t486-Ii_31.*t3.*t4.*t210.*t485+...
         Ii_32.*t2.*t5.*t209.*t485.*(1.0./2.0)+Ii_31.*t2.*t5.*t210.*t486-Ii_31.*t3.*t5.*t210.*t485+Ii_32.*t3.*t4.*t209.*t486.*(1.0./2.0)+...
         Ii_32.*t3.*t5.*t209.*t486.*(1.0./2.0)-Ii_11.*t4.*t118.*t206.*t488.*(1.0./8.0)-...
         Ii_11.*t5.*t118.*t206.*t488.*(1.0./8.0)-Ii_21.*t4.*t118.*t205.*t487-Ii_21.*t5.*t118.*t205.*t487+Ii_22.*t4.*t118.*t205.*t488.*(1.0./4.0)+...
         Ii_22.*t5.*t118.*t205.*t488.*(1.0./4.0)+Ii_11.*t23.*t118.*t205.*t488.*(1.0./4.0)-...
         Ii_33.*t4.*t118.*t205.*t488.*(1.0./4.0)+Ii_33.*t4.*t118.*t206.*t488.*(1.0./8.0)-Ii_33.*t5.*t118.*t205.*t488.*(1.0./4.0)-...
         Ii_31.*t4.*t118.*t209.*t488.*(1.0./4.0)+Ii_32.*t4.*t118.*t209.*t487+Ii_33.*t5.*t118.*t206.*t488.*(1.0./8.0)+Ii_31.*t4.*t118.*t210.*t488.*(1.0./4.0)-...
         Ii_31.*t5.*t118.*t209.*t488.*(1.0./4.0)+Ii_32.*t5.*t118.*t209.*t487+Ii_31.*t5.*t118.*t210.*t488.*(1.0./4.0)-...
         Ii_33.*t23.*t118.*t205.*t488.*(1.0./4.0)-Ii_31.*t23.*t118.*t209.*t488.*(1.0./2.0)-Ii_11.*t2.*t4.*t486.*t490.*(1.0./4.0)+...
         Ii_11.*t3.*t4.*t485.*t490.*(1.0./4.0)-Ii_11.*t2.*t5.*t486.*t490.*(1.0./4.0)+Ii_11.*t3.*t5.*t485.*t490.*(1.0./4.0)-...
         Ii_11.*t2.*t4.*t486.*t493.*(1.0./4.0)+Ii_11.*t3.*t4.*t485.*t493.*(1.0./4.0)-Ii_11.*t2.*t5.*t486.*t493.*(1.0./4.0)+...
         Ii_11.*t3.*t5.*t485.*t493.*(1.0./4.0)+Ii_21.*t2.*t4.*t485.*t490.*(1.0./4.0)+...
         Ii_21.*t2.*t5.*t485.*t490.*(1.0./4.0)+Ii_21.*t3.*t4.*t486.*t490.*(1.0./4.0)-Ii_21.*t2.*t4.*t485.*t493.*(3.0./4.0)+...
         Ii_21.*t3.*t5.*t486.*t490.*(1.0./4.0)-Ii_21.*t2.*t5.*t485.*t493.*(3.0./4.0)-Ii_21.*t3.*t4.*t486.*t493.*(3.0./4.0)-Ii_21.*t3.*t5.*t486.*t493.*(3.0./4.0)+...
         Ii_31.*t2.*t4.*t486.*t491.*(1.0./2.0)-Ii_31.*t3.*t4.*t485.*t491.*(1.0./2.0)+Ii_32.*t2.*t4.*t485.*t491.*(1.0./4.0)+Ii_31.*t2.*t4.*t486.*t492.*(1.0./2.0)+...
         Ii_31.*t2.*t5.*t486.*t491.*(1.0./2.0)-Ii_31.*t3.*t4.*t485.*t492.*(1.0./2.0)-Ii_31.*t3.*t5.*t485.*t491.*(1.0./2.0)+Ii_32.*t2.*t4.*t485.*t492.*(3.0./4.0)+...
         Ii_32.*t2.*t5.*t485.*t491.*(1.0./4.0)+Ii_33.*t2.*t4.*t486.*t490.*(1.0./4.0)-Ii_33.*t3.*t4.*t485.*t490.*(1.0./4.0)+Ii_31.*t2.*t5.*t486.*t492.*(1.0./2.0)-...
         Ii_31.*t3.*t5.*t485.*t492.*(1.0./2.0)+Ii_32.*t2.*t5.*t485.*t492.*(3.0./4.0)+Ii_32.*t3.*t4.*t486.*t491.*(1.0./4.0)+Ii_33.*t2.*t5.*t486.*t490.*(1.0./4.0)-...
         Ii_33.*t3.*t5.*t485.*t490.*(1.0./4.0)+Ii_32.*t3.*t4.*t486.*t492.*(3.0./4.0)+Ii_32.*t3.*t5.*t486.*t491.*(1.0./4.0)+Ii_32.*t3.*t5.*t486.*t492.*(3.0./4.0)+...
         Ii_33.*t2.*t4.*t486.*t493.*(1.0./4.0)-Ii_33.*t3.*t4.*t485.*t493.*(1.0./4.0)+Ii_33.*t2.*t5.*t486.*t493.*(1.0./4.0)-Ii_33.*t3.*t5.*t485.*t493.*(1.0./4.0)-...
         Ii_11.*t4.*t118.*t488.*t490.*(1.0./4.0)-Ii_11.*t5.*t118.*t488.*t490.*(1.0./4.0)-Ii_11.*t4.*t118.*t488.*t493.*(1.0./4.0)-Ii_11.*t5.*t118.*t488.*t493.*(1.0./4.0)+...
         Ii_21.*t4.*t118.*t487.*t490.*(1.0./8.0)+Ii_21.*t5.*t118.*t487.*t490.*(1.0./8.0)+Ii_22.*t4.*t118.*t488.*t490-Ii_21.*t4.*t118.*t487.*t493.*(3.0./8.0)+Ii_22.*t5.*t118.*t488.*t490-...
         Ii_21.*t5.*t118.*t487.*t493.*(3.0./8.0)-Ii_31.*t4.*t118.*t488.*t491.*(1.0./2.0)-Ii_32.*t4.*t118.*t487.*t491.*(3.0./8.0)+Ii_31.*t4.*t118.*t488.*t492.*(1.0./2.0)-...
         Ii_31.*t5.*t118.*t488.*t491.*(1.0./2.0)+Ii_32.*t4.*t118.*t487.*t492.*(3.0./8.0)-Ii_32.*t5.*t118.*t487.*t491.*(3.0./8.0)-Ii_33.*t4.*t118.*t488.*t490.*(3.0./4.0)+...
         Ii_31.*t5.*t118.*t488.*t492.*(1.0./2.0)+Ii_32.*t5.*t118.*t487.*t492.*(3.0./8.0)-Ii_33.*t5.*t118.*t488.*t490.*(3.0./4.0)+Ii_33.*t4.*t118.*t488.*t493.*(1.0./4.0)+...
         Ii_33.*t5.*t118.*t488.*t493.*(1.0./4.0)+Ii_21.*t23.*t118.*t487.*t490.*(1.0./2.0)-Ii_32.*t23.*t118.*t487.*t491.*(1.0./2.0)+Ii_11.*t4.*t206.*t487.*t489.*(1.0./8.0)+...
         Ii_11.*t5.*t206.*t487.*t489.*(1.0./8.0)-Ii_21.*t4.*t205.*t488.*t489-Ii_22.*t4.*t205.*t487.*t489.*(1.0./4.0)-Ii_21.*t5.*t205.*t488.*t489-Ii_22.*t5.*t205.*t487.*t489.*(1.0./4.0)-...
         Ii_11.*t23.*t205.*t487.*t489.*(1.0./4.0)+Ii_33.*t4.*t205.*t487.*t489.*(1.0./4.0)-Ii_33.*t4.*t206.*t487.*t489.*(1.0./8.0)+Ii_33.*t5.*t205.*t487.*t489.*(1.0./4.0)+...
         Ii_31.*t4.*t209.*t487.*t489.*(1.0./4.0)-Ii_33.*t5.*t206.*t487.*t489.*(1.0./8.0)-Ii_31.*t4.*t210.*t487.*t489.*(1.0./4.0)+Ii_31.*t5.*t209.*t487.*t489.*(1.0./4.0)-...
         Ii_31.*t5.*t210.*t487.*t489.*(1.0./4.0)+Ii_32.*t4.*t209.*t488.*t489+Ii_32.*t5.*t209.*t488.*t489+Ii_33.*t23.*t205.*t487.*t489.*(1.0./4.0)+Ii_31.*t23.*t209.*t487.*t489.*(1.0./2.0)+...
         Ii_11.*t4.*t487.*t489.*t490.*(1.0./4.0)+Ii_11.*t5.*t487.*t489.*t490.*(1.0./4.0)+Ii_11.*t4.*t487.*t489.*t493.*(1.0./4.0)+Ii_11.*t5.*t487.*t489.*t493.*(1.0./4.0)+...
         Ii_21.*t4.*t488.*t489.*t490.*(1.0./8.0)-Ii_22.*t4.*t487.*t489.*t490+Ii_21.*t5.*t488.*t489.*t490.*(1.0./8.0)-Ii_22.*t5.*t487.*t489.*t490-Ii_21.*t4.*t488.*t489.*t493.*(3.0./8.0)-...
         Ii_21.*t5.*t488.*t489.*t493.*(3.0./8.0)+Ii_31.*t4.*t487.*t489.*t491.*(1.0./2.0)-Ii_31.*t4.*t487.*t489.*t492.*(1.0./2.0)+Ii_31.*t5.*t487.*t489.*t491.*(1.0./2.0)+...
         Ii_33.*t4.*t487.*t489.*t490.*(3.0./4.0)-Ii_31.*t5.*t487.*t489.*t492.*(1.0./2.0)-Ii_32.*t4.*t488.*t489.*t491.*(3.0./8.0)+Ii_33.*t5.*t487.*t489.*t490.*(3.0./4.0)+...
         Ii_32.*t4.*t488.*t489.*t492.*(3.0./8.0)-Ii_32.*t5.*t488.*t489.*t491.*(3.0./8.0)+Ii_32.*t5.*t488.*t489.*t492.*(3.0./8.0)-Ii_33.*t4.*t487.*t489.*t493.*(1.0./4.0)-...
         Ii_33.*t5.*t487.*t489.*t493.*(1.0./4.0)+Ii_21.*t23.*t488.*t489.*t490.*(1.0./2.0)-Ii_32.*t23.*t488.*t489.*t491.*(1.0./2.0)-Ii_11.*deltap_i.*phip_i.*t118.*t209.*t487.*(1.0./2.0)-...
         Ii_31.*deltap_i.*phip_i.*t118.*t205.*t487+Ii_33.*deltap_i.*phip_i.*t118.*t209.*t487.*(1.0./2.0)+Ii_21.*deltap_i.*phip_i.*t118.*t488.*t491.*2.0+Ii_32.*deltap_i.*phip_i.*t118.*t488.*t490.*2.0-...
         Ii_11.*deltap_i.*phip_i.*t209.*t488.*t489.*(1.0./2.0)-Ii_31.*deltap_i.*phip_i.*t205.*t488.*t489+Ii_33.*deltap_i.*phip_i.*t209.*t488.*t489.*(1.0./2.0)-Ii_21.*deltap_i.*phip_i.*t487.*t489.*t491.*2.0-...
         Ii_32.*deltap_i.*phip_i.*t487.*t489.*t490.*2.0-Ii_11.*deltap_i.*t2.*t206.*t486.*thetap+Ii_11.*deltap_i.*t3.*t206.*t485.*thetap-Ii_21.*deltap_i.*t2.*t205.*t485.*thetap-...
         Ii_21.*deltap_i.*t3.*t205.*t486.*thetap+Ii_33.*deltap_i.*t2.*t206.*t486.*thetap-...
         Ii_33.*deltap_i.*t3.*t206.*t485.*thetap+Ii_32.*deltap_i.*t2.*t209.*t485.*thetap+Ii_31.*deltap_i.*t2.*t210.*t486.*thetap.*2.0-Ii_31.*deltap_i.*t3.*t210.*t485.*thetap.*2.0+...
         Ii_32.*deltap_i.*t3.*t209.*t486.*thetap-Ii_11.*deltap_i.*t118.*t206.*t488.*thetap.*(1.0./4.0)-Ii_21.*deltap_i.*t118.*t205.*t487.*thetap.*2.0+Ii_22.*deltap_i.*t118.*t205.*t488.*thetap.*(1.0./2.0)-...
         Ii_33.*deltap_i.*t118.*t205.*t488.*thetap.*(1.0./2.0)+Ii_33.*deltap_i.*t118.*t206.*t488.*thetap.*(1.0./4.0)-Ii_31.*deltap_i.*t118.*t209.*t488.*thetap.*(1.0./2.0)+...
         Ii_32.*deltap_i.*t118.*t209.*t487.*thetap.*2.0+Ii_31.*deltap_i.*t118.*t210.*t488.*thetap.*(1.0./2.0)-Ii_11.*deltap_i.*t2.*t486.*t490.*thetap.*(1.0./2.0)+...
         Ii_11.*deltap_i.*t3.*t485.*t490.*thetap.*(1.0./2.0)-Ii_11.*deltap_i.*t2.*t486.*t493.*thetap.*(1.0./2.0)+Ii_11.*deltap_i.*t3.*t485.*t493.*thetap.*(1.0./2.0)+Ii_21.*deltap_i.*t2.*t485.*t490.*thetap.*(1.0./2.0)+...
         Ii_21.*deltap_i.*t3.*t486.*t490.*thetap.*(1.0./2.0)-Ii_21.*deltap_i.*t2.*t485.*t493.*thetap.*(3.0./2.0)-Ii_21.*deltap_i.*t3.*t486.*t493.*thetap.*(3.0./2.0)+Ii_31.*deltap_i.*t2.*t486.*t491.*thetap-...
         Ii_31.*deltap_i.*t3.*t485.*t491.*thetap+Ii_32.*deltap_i.*t2.*t485.*t491.*thetap.*(1.0./2.0)+Ii_31.*deltap_i.*t2.*t486.*t492.*thetap-Ii_31.*deltap_i.*t3.*t485.*t492.*thetap+...
         Ii_32.*deltap_i.*t2.*t485.*t492.*thetap.*(3.0./2.0)+Ii_33.*deltap_i.*t2.*t486.*t490.*thetap.*(1.0./2.0)-Ii_33.*deltap_i.*t3.*t485.*t490.*thetap.*(1.0./2.0)+Ii_32.*deltap_i.*t3.*t486.*t491.*thetap.*(1.0./2.0)+...
         Ii_32.*deltap_i.*t3.*t486.*t492.*thetap.*(3.0./2.0)+Ii_33.*deltap_i.*t2.*t486.*t493.*thetap.*(1.0./2.0)-Ii_33.*deltap_i.*t3.*t485.*t493.*thetap.*(1.0./2.0)-Ii_11.*deltap_i.*t118.*t488.*t490.*thetap.*(1.0./2.0)-...
         Ii_11.*deltap_i.*t118.*t488.*t493.*thetap.*(1.0./2.0)+Ii_21.*deltap_i.*t118.*t487.*t490.*thetap.*(1.0./4.0)+Ii_22.*deltap_i.*t118.*t488.*t490.*thetap.*2.0-Ii_21.*deltap_i.*t118.*t487.*t493.*thetap.*(3.0./4.0)-...
         Ii_31.*deltap_i.*t118.*t488.*t491.*thetap-Ii_32.*deltap_i.*t118.*t487.*t491.*thetap.*(3.0./4.0)+Ii_31.*deltap_i.*t118.*t488.*t492.*thetap+Ii_32.*deltap_i.*t118.*t487.*t492.*thetap.*(3.0./4.0)-...
         Ii_33.*deltap_i.*t118.*t488.*t490.*thetap.*(3.0./2.0)+Ii_33.*deltap_i.*t118.*t488.*t493.*thetap.*(1.0./2.0)+Ii_11.*deltap_i.*t206.*t487.*t489.*thetap.*(1.0./4.0)-...
         Ii_21.*deltap_i.*t205.*t488.*t489.*thetap.*2.0-Ii_22.*deltap_i.*t205.*t487.*t489.*thetap.*(1.0./2.0)+Ii_33.*deltap_i.*t205.*t487.*t489.*thetap.*(1.0./2.0)-...
         Ii_33.*deltap_i.*t206.*t487.*t489.*thetap.*(1.0./4.0)+Ii_31.*deltap_i.*t209.*t487.*t489.*thetap.*(1.0./2.0)-Ii_31.*deltap_i.*t210.*t487.*t489.*thetap.*(1.0./2.0)+...
         Ii_32.*deltap_i.*t209.*t488.*t489.*thetap.*2.0+Ii_11.*deltap_i.*t487.*t489.*t490.*thetap.*(1.0./2.0)+Ii_11.*deltap_i.*t487.*t489.*t493.*thetap.*(1.0./2.0)+...
         Ii_21.*deltap_i.*t488.*t489.*t490.*thetap.*(1.0./4.0)-Ii_22.*deltap_i.*t487.*t489.*t490.*thetap.*2.0-Ii_21.*deltap_i.*t488.*t489.*t493.*thetap.*(3.0./4.0)+...
         Ii_31.*deltap_i.*t487.*t489.*t491.*thetap-Ii_31.*deltap_i.*t487.*t489.*t492.*thetap+Ii_33.*deltap_i.*t487.*t489.*t490.*thetap.*(3.0./2.0)-Ii_32.*deltap_i.*t488.*t489.*t491.*thetap.*(3.0./4.0)+...
         Ii_32.*deltap_i.*t488.*t489.*t492.*thetap.*(3.0./4.0)-Ii_33.*deltap_i.*t487.*t489.*t493.*thetap.*(1.0./2.0)-Ii_11.*phip_i.*t118.*t209.*t487.*thetap.*(1.0./2.0)-Ii_31.*phip_i.*t118.*t205.*t487.*thetap+...
         Ii_33.*phip_i.*t118.*t209.*t487.*thetap.*(1.0./2.0)+Ii_21.*phip_i.*t118.*t488.*t491.*thetap.*2.0+Ii_32.*phip_i.*t118.*t488.*t490.*thetap.*2.0-...
         Ii_11.*phip_i.*t209.*t488.*t489.*thetap.*(1.0./2.0)-Ii_31.*phip_i.*t205.*t488.*t489.*thetap+Ii_33.*phip_i.*t209.*t488.*t489.*thetap.*(1.0./2.0)-...
         Ii_21.*phip_i.*t487.*t489.*t491.*thetap.*2.0-Ii_32.*phip_i.*t487.*t489.*t490.*thetap.*2.0;
    
    Q71 = f_phi_o+Io_11.*t4.*t208.*(3.0./8.0)+Io_11.*t8.*t208.*(3.0./8.0)+Io_22.*t4.*t207.*(1.0./4.0)+Io_22.*t8.*t207.*(1.0./4.0)-Io_33.*t4.*t207.*(1.0./4.0)+...
         Io_11.*t27.*t207.*(1.0./4.0)-Io_33.*t4.*t208.*(3.0./8.0)-Io_31.*t4.*t211.*(1.0./4.0)-Io_31.*t4.*t212.*(3.0./4.0)-Io_33.*t8.*t207.*(1.0./4.0)-...
         Io_33.*t8.*t208.*(3.0./8.0)-Io_31.*t8.*t211.*(1.0./4.0)-Io_31.*t8.*t212.*(3.0./4.0)-Io_33.*t27.*t207.*(1.0./4.0)-Io_31.*t27.*t211.*(1.0./2.0)+...
         Io_32.*t2.*t4.*t494.*(1.0./2.0)+Io_32.*t3.*t4.*t495.*(1.0./2.0)+Io_32.*t2.*t8.*t494.*(1.0./2.0)+Io_32.*t3.*t8.*t495.*(1.0./2.0)-Io_32.*t4.*t118.*t496-...
         Io_32.*t8.*t118.*t496-Io_32.*t4.*t489.*t497-Io_32.*t8.*t489.*t497+Io_11.*deltap_o.*t208.*thetap.*(3.0./4.0)+Io_22.*deltap_o.*t207.*thetap.*(1.0./2.0)-...
         Io_33.*deltap_o.*t207.*thetap.*(1.0./2.0)-Io_33.*deltap_o.*t208.*thetap.*(3.0./4.0)-Io_31.*deltap_o.*t211.*thetap.*(1.0./2.0)-Io_31.*deltap_o.*t212.*thetap.*(3.0./2.0)-...
         Io_11.*deltap_o.*phip_o.*t118.*t496.*(1.0./2.0)+Io_22.*deltap_o.*phip_o.*t118.*t496-Io_33.*deltap_o.*phip_o.*t118.*t496.*(1.0./2.0)-Io_11.*deltap_o.*phip_o.*t489.*t497.*(1.0./2.0)+...
         Io_22.*deltap_o.*phip_o.*t489.*t497-Io_33.*deltap_o.*phip_o.*t489.*t497.*(1.0./2.0)+Io_32.*deltap_o.*t2.*t494.*thetap+Io_32.*deltap_o.*t3.*t495.*thetap-Io_32.*deltap_o.*t118.*t496.*thetap.*2.0-...
         Io_32.*deltap_o.*t489.*t497.*thetap.*2.0-Io_11.*phip_o.*t118.*t496.*thetap.*(1.0./2.0)+Io_22.*phip_o.*t118.*t496.*thetap-Io_33.*phip_o.*t118.*t496.*thetap.*(1.0./2.0)-...
         Io_11.*phip_o.*t489.*t497.*thetap.*(1.0./2.0)+Io_22.*phip_o.*t489.*t497.*thetap-Io_33.*phip_o.*t489.*t497.*thetap.*(1.0./2.0)-Io_11.*t2.*t4.*t208.*t495.*(1.0./2.0)+...
         Io_11.*t3.*t4.*t208.*t494.*(1.0./2.0)-Io_11.*t2.*t8.*t208.*t495.*(1.0./2.0)+Io_11.*t3.*t8.*t208.*t494.*(1.0./2.0)-Io_21.*t2.*t4.*t207.*t494.*(1.0./2.0)-Io_21.*t3.*t4.*t207.*t495.*(1.0./2.0)-...
         Io_21.*t2.*t8.*t207.*t494.*(1.0./2.0)-Io_21.*t3.*t8.*t207.*t495.*(1.0./2.0)+Io_33.*t2.*t4.*t208.*t495.*(1.0./2.0)-Io_33.*t3.*t4.*t208.*t494.*(1.0./2.0)+Io_32.*t2.*t4.*t211.*t494.*(1.0./2.0)+...
         Io_31.*t2.*t4.*t212.*t495-Io_31.*t3.*t4.*t212.*t494+Io_32.*t3.*t4.*t211.*t495.*(1.0./2.0)+Io_33.*t2.*t8.*t208.*t495.*(1.0./2.0)-Io_33.*t3.*t8.*t208.*t494.*(1.0./2.0)+...
         Io_32.*t2.*t8.*t211.*t494.*(1.0./2.0)+Io_31.*t2.*t8.*t212.*t495-Io_31.*t3.*t8.*t212.*t494+Io_32.*t3.*t8.*t211.*t495.*(1.0./2.0)-Io_11.*t4.*t118.*t208.*t497.*(1.0./8.0)-...
         Io_11.*t8.*t118.*t208.*t497.*(1.0./8.0)-Io_21.*t4.*t118.*t207.*t496+Io_22.*t4.*t118.*t207.*t497.*(1.0./4.0)-Io_21.*t8.*t118.*t207.*t496+Io_22.*t8.*t118.*t207.*t497.*(1.0./4.0)-...
         Io_33.*t4.*t118.*t207.*t497.*(1.0./4.0)+Io_11.*t27.*t118.*t207.*t497.*(1.0./4.0)+Io_33.*t4.*t118.*t208.*t497.*(1.0./8.0)-Io_31.*t4.*t118.*t211.*t497.*(1.0./4.0)+Io_32.*t4.*t118.*t211.*t496+...
         Io_31.*t4.*t118.*t212.*t497.*(1.0./4.0)-Io_33.*t8.*t118.*t207.*t497.*(1.0./4.0)+Io_33.*t8.*t118.*t208.*t497.*(1.0./8.0)-Io_31.*t8.*t118.*t211.*t497.*(1.0./4.0)+Io_32.*t8.*t118.*t211.*t496+...
         Io_31.*t8.*t118.*t212.*t497.*(1.0./4.0)-Io_33.*t27.*t118.*t207.*t497.*(1.0./4.0)-Io_31.*t27.*t118.*t211.*t497.*(1.0./2.0)-Io_11.*t2.*t4.*t495.*t498.*(1.0./4.0)+...
         Io_11.*t3.*t4.*t494.*t498.*(1.0./4.0)-Io_11.*t2.*t4.*t495.*t501.*(1.0./4.0)+Io_11.*t3.*t4.*t494.*t501.*(1.0./4.0)-Io_11.*t2.*t8.*t495.*t498.*(1.0./4.0)+...
         Io_11.*t3.*t8.*t494.*t498.*(1.0./4.0)-Io_11.*t2.*t8.*t495.*t501.*(1.0./4.0)+Io_11.*t3.*t8.*t494.*t501.*(1.0./4.0)+Io_21.*t2.*t4.*t494.*t498.*(1.0./4.0)+...
         Io_21.*t3.*t4.*t495.*t498.*(1.0./4.0)-Io_21.*t2.*t4.*t494.*t501.*(3.0./4.0)+Io_21.*t2.*t8.*t494.*t498.*(1.0./4.0)-Io_21.*t3.*t4.*t495.*t501.*(3.0./4.0)+...
         Io_21.*t3.*t8.*t495.*t498.*(1.0./4.0)-Io_21.*t2.*t8.*t494.*t501.*(3.0./4.0)-Io_21.*t3.*t8.*t495.*t501.*(3.0./4.0)+Io_31.*t2.*t4.*t495.*t499.*(1.0./2.0)-...
         Io_31.*t3.*t4.*t494.*t499.*(1.0./2.0)+Io_32.*t2.*t4.*t494.*t499.*(1.0./4.0)+Io_31.*t2.*t4.*t495.*t500.*(1.0./2.0)-Io_31.*t3.*t4.*t494.*t500.*(1.0./2.0)+...
         Io_32.*t2.*t4.*t494.*t500.*(3.0./4.0)+Io_33.*t2.*t4.*t495.*t498.*(1.0./4.0)-Io_33.*t3.*t4.*t494.*t498.*(1.0./4.0)+Io_32.*t3.*t4.*t495.*t499.*(1.0./4.0)+...
         Io_32.*t3.*t4.*t495.*t500.*(3.0./4.0)+Io_31.*t2.*t8.*t495.*t499.*(1.0./2.0)-Io_31.*t3.*t8.*t494.*t499.*(1.0./2.0)+Io_32.*t2.*t8.*t494.*t499.*(1.0./4.0)+...
         Io_33.*t2.*t4.*t495.*t501.*(1.0./4.0)-Io_33.*t3.*t4.*t494.*t501.*(1.0./4.0)+Io_31.*t2.*t8.*t495.*t500.*(1.0./2.0)-Io_31.*t3.*t8.*t494.*t500.*(1.0./2.0)+...
         Io_32.*t2.*t8.*t494.*t500.*(3.0./4.0)+Io_33.*t2.*t8.*t495.*t498.*(1.0./4.0)-Io_33.*t3.*t8.*t494.*t498.*(1.0./4.0)+Io_32.*t3.*t8.*t495.*t499.*(1.0./4.0)+...
         Io_32.*t3.*t8.*t495.*t500.*(3.0./4.0)+Io_33.*t2.*t8.*t495.*t501.*(1.0./4.0)-Io_33.*t3.*t8.*t494.*t501.*(1.0./4.0)-Io_11.*t4.*t118.*t497.*t498.*(1.0./4.0)-...
         Io_11.*t4.*t118.*t497.*t501.*(1.0./4.0)-Io_11.*t8.*t118.*t497.*t498.*(1.0./4.0)-Io_11.*t8.*t118.*t497.*t501.*(1.0./4.0)+Io_21.*t4.*t118.*t496.*t498.*(1.0./8.0)+...
         Io_22.*t4.*t118.*t497.*t498-Io_21.*t4.*t118.*t496.*t501.*(3.0./8.0)+Io_21.*t8.*t118.*t496.*t498.*(1.0./8.0)+Io_22.*t8.*t118.*t497.*t498-...
         Io_21.*t8.*t118.*t496.*t501.*(3.0./8.0)-Io_31.*t4.*t118.*t497.*t499.*(1.0./2.0)-Io_32.*t4.*t118.*t496.*t499.*(3.0./8.0)+Io_31.*t4.*t118.*t497.*t500.*(1.0./2.0)+...
         Io_32.*t4.*t118.*t496.*t500.*(3.0./8.0)-Io_33.*t4.*t118.*t497.*t498.*(3.0./4.0)-Io_31.*t8.*t118.*t497.*t499.*(1.0./2.0)-Io_32.*t8.*t118.*t496.*t499.*(3.0./8.0)+...
         Io_33.*t4.*t118.*t497.*t501.*(1.0./4.0)+Io_31.*t8.*t118.*t497.*t500.*(1.0./2.0)+Io_32.*t8.*t118.*t496.*t500.*(3.0./8.0)-Io_33.*t8.*t118.*t497.*t498.*(3.0./4.0)+...
         Io_33.*t8.*t118.*t497.*t501.*(1.0./4.0)+...
         Io_21.*t27.*t118.*t496.*t498.*(1.0./2.0)-Io_32.*t27.*t118.*t496.*t499.*(1.0./2.0)+Io_11.*t4.*t208.*t489.*t496.*(1.0./8.0)+Io_11.*t8.*t208.*t489.*t496.*(1.0./8.0)-...
         Io_21.*t4.*t207.*t489.*t497-Io_22.*t4.*t207.*t489.*t496.*(1.0./4.0)-Io_21.*t8.*t207.*t489.*t497-Io_22.*t8.*t207.*t489.*t496.*(1.0./4.0)+...
         Io_33.*t4.*t207.*t489.*t496.*(1.0./4.0)-Io_11.*t27.*t207.*t489.*t496.*(1.0./4.0)-Io_33.*t4.*t208.*t489.*t496.*(1.0./8.0)+...
         Io_31.*t4.*t211.*t489.*t496.*(1.0./4.0)-Io_31.*t4.*t212.*t489.*t496.*(1.0./4.0)+Io_32.*t4.*t211.*t489.*t497+Io_33.*t8.*t207.*t489.*t496.*(1.0./4.0)-...
         Io_33.*t8.*t208.*t489.*t496.*(1.0./8.0)+Io_31.*t8.*t211.*t489.*t496.*(1.0./4.0)-Io_31.*t8.*t212.*t489.*t496.*(1.0./4.0)+Io_32.*t8.*t211.*t489.*t497+...
         Io_33.*t27.*t207.*t489.*t496.*(1.0./4.0)+Io_31.*t27.*t211.*t489.*t496.*(1.0./2.0)+Io_11.*t4.*t489.*t496.*t498.*(1.0./4.0)+Io_11.*t4.*t489.*t496.*t501.*(1.0./4.0)+...
         Io_11.*t8.*t489.*t496.*t498.*(1.0./4.0)+Io_11.*t8.*t489.*t496.*t501.*(1.0./4.0)+Io_21.*t4.*t489.*t497.*t498.*(1.0./8.0)-Io_22.*t4.*t489.*t496.*t498-...
         Io_21.*t4.*t489.*t497.*t501.*(3.0./8.0)+Io_21.*t8.*t489.*t497.*t498.*(1.0./8.0)-Io_22.*t8.*t489.*t496.*t498-Io_21.*t8.*t489.*t497.*t501.*(3.0./8.0)+...
         Io_31.*t4.*t489.*t496.*t499.*(1.0./2.0)-Io_31.*t4.*t489.*t496.*t500.*(1.0./2.0)+Io_33.*t4.*t489.*t496.*t498.*(3.0./4.0)-Io_32.*t4.*t489.*t497.*t499.*(3.0./8.0)+...
         Io_32.*t4.*t489.*t497.*t500.*(3.0./8.0)+Io_31.*t8.*t489.*t496.*t499.*(1.0./2.0)-Io_33.*t4.*t489.*t496.*t501.*(1.0./4.0)-Io_31.*t8.*t489.*t496.*t500.*(1.0./2.0)+...
         Io_33.*t8.*t489.*t496.*t498.*(3.0./4.0)-Io_32.*t8.*t489.*t497.*t499.*(3.0./8.0)+Io_32.*t8.*t489.*t497.*t500.*(3.0./8.0)-Io_33.*t8.*t489.*t496.*t501.*(1.0./4.0)+...
         Io_21.*t27.*t489.*t497.*t498.*(1.0./2.0)-Io_32.*t27.*t489.*t497.*t499.*(1.0./2.0)-Io_11.*deltap_o.*phip_o.*t118.*t211.*t496.*(1.0./2.0)-Io_31.*deltap_o.*phip_o.*t118.*t207.*t496+...
         Io_33.*deltap_o.*phip_o.*t118.*t211.*t496.*(1.0./2.0)+Io_21.*deltap_o.*phip_o.*t118.*t497.*t499.*2.0+Io_32.*deltap_o.*phip_o.*t118.*t497.*t498.*2.0-...
         Io_11.*deltap_o.*phip_o.*t211.*t489.*t497.*(1.0./2.0)-Io_31.*deltap_o.*phip_o.*t207.*t489.*t497+Io_33.*deltap_o.*phip_o.*t211.*t489.*t497.*(1.0./2.0)-...
         Io_21.*deltap_o.*phip_o.*t489.*t496.*t499.*2.0-Io_32.*deltap_o.*phip_o.*t489.*t496.*t498.*2.0-Io_11.*deltap_o.*t2.*t208.*t495.*thetap+Io_11.*deltap_o.*t3.*t208.*t494.*thetap-...
         Io_21.*deltap_o.*t2.*t207.*t494.*thetap-Io_21.*deltap_o.*t3.*t207.*t495.*thetap+Io_33.*deltap_o.*t2.*t208.*t495.*thetap-Io_33.*deltap_o.*t3.*t208.*t494.*thetap+...
         Io_32.*deltap_o.*t2.*t211.*t494.*thetap+Io_31.*deltap_o.*t2.*t212.*t495.*thetap.*2.0-Io_31.*deltap_o.*t3.*t212.*t494.*thetap.*2.0+Io_32.*deltap_o.*t3.*t211.*t495.*thetap-...
         Io_11.*deltap_o.*t118.*t208.*t497.*thetap.*(1.0./4.0)-Io_21.*deltap_o.*t118.*t207.*t496.*thetap.*2.0+Io_22.*deltap_o.*t118.*t207.*t497.*thetap.*(1.0./2.0)-...
         Io_33.*deltap_o.*t118.*t207.*t497.*thetap.*(1.0./2.0)+Io_33.*deltap_o.*t118.*t208.*t497.*thetap.*(1.0./4.0)-Io_31.*deltap_o.*t118.*t211.*t497.*thetap.*(1.0./2.0)+...
         Io_32.*deltap_o.*t118.*t211.*t496.*thetap.*2.0+Io_31.*deltap_o.*t118.*t212.*t497.*thetap.*(1.0./2.0)-Io_11.*deltap_o.*t2.*t495.*t498.*thetap.*(1.0./2.0)+...
         Io_11.*deltap_o.*t3.*t494.*t498.*thetap.*(1.0./2.0)-Io_11.*deltap_o.*t2.*t495.*t501.*thetap.*(1.0./2.0)+Io_11.*deltap_o.*t3.*t494.*t501.*thetap.*(1.0./2.0)+...
         Io_21.*deltap_o.*t2.*t494.*t498.*thetap.*(1.0./2.0)+Io_21.*deltap_o.*t3.*t495.*t498.*thetap.*(1.0./2.0)-Io_21.*deltap_o.*t2.*t494.*t501.*thetap.*(3.0./2.0)-...
         Io_21.*deltap_o.*t3.*t495.*t501.*thetap.*(3.0./2.0)+Io_31.*deltap_o.*t2.*t495.*t499.*thetap-Io_31.*deltap_o.*t3.*t494.*t499.*thetap+...
         Io_32.*deltap_o.*t2.*t494.*t499.*thetap.*(1.0./2.0)+Io_31.*deltap_o.*t2.*t495.*t500.*thetap-Io_31.*deltap_o.*t3.*t494.*t500.*thetap+Io_32.*deltap_o.*t2.*t494.*t500.*thetap.*(3.0./2.0)+...
         Io_33.*deltap_o.*t2.*t495.*t498.*thetap.*(1.0./2.0)-Io_33.*deltap_o.*t3.*t494.*t498.*thetap.*(1.0./2.0)+Io_32.*deltap_o.*t3.*t495.*t499.*thetap.*(1.0./2.0)+...
         Io_32.*deltap_o.*t3.*t495.*t500.*thetap.*(3.0./2.0)+Io_33.*deltap_o.*t2.*t495.*t501.*thetap.*(1.0./2.0)-Io_33.*deltap_o.*t3.*t494.*t501.*thetap.*(1.0./2.0)-...
         Io_11.*deltap_o.*t118.*t497.*t498.*thetap.*(1.0./2.0)-Io_11.*deltap_o.*t118.*t497.*t501.*thetap.*(1.0./2.0)+Io_21.*deltap_o.*t118.*t496.*t498.*thetap.*(1.0./4.0)+...
         Io_22.*deltap_o.*t118.*t497.*t498.*thetap.*2.0-Io_21.*deltap_o.*t118.*t496.*t501.*thetap.*(3.0./4.0)-Io_31.*deltap_o.*t118.*t497.*t499.*thetap-...
         Io_32.*deltap_o.*t118.*t496.*t499.*thetap.*(3.0./4.0)+Io_31.*deltap_o.*t118.*t497.*t500.*thetap+Io_32.*deltap_o.*t118.*t496.*t500.*thetap.*(3.0./4.0)-...
         Io_33.*deltap_o.*t118.*t497.*t498.*thetap.*(3.0./2.0)+Io_33.*deltap_o.*t118.*t497.*t501.*thetap.*(1.0./2.0)+...
         Io_11.*deltap_o.*t208.*t489.*t496.*thetap.*(1.0./4.0)-...
         Io_21.*deltap_o.*t207.*t489.*t497.*thetap.*2.0-Io_22.*deltap_o.*t207.*t489.*t496.*thetap.*(1.0./2.0)+...
         Io_33.*deltap_o.*t207.*t489.*t496.*thetap.*(1.0./2.0)-Io_33.*deltap_o.*t208.*t489.*t496.*thetap.*(1.0./4.0)+...
         Io_31.*deltap_o.*t211.*t489.*t496.*thetap.*(1.0./2.0)-Io_31.*deltap_o.*t212.*t489.*t496.*thetap.*(1.0./2.0)+...
         Io_32.*deltap_o.*t211.*t489.*t497.*thetap.*2.0+Io_11.*deltap_o.*t489.*t496.*t498.*thetap.*(1.0./2.0)+...
         Io_11.*deltap_o.*t489.*t496.*t501.*thetap.*(1.0./2.0)+Io_21.*deltap_o.*t489.*t497.*t498.*thetap.*(1.0./4.0)-...
         Io_22.*deltap_o.*t489.*t496.*t498.*thetap.*2.0-Io_21.*deltap_o.*t489.*t497.*t501.*thetap.*(3.0./4.0)+...
         Io_31.*deltap_o.*t489.*t496.*t499.*thetap-Io_31.*deltap_o.*t489.*t496.*t500.*thetap+...
         Io_33.*deltap_o.*t489.*t496.*t498.*thetap.*(3.0./2.0)-Io_32.*deltap_o.*t489.*t497.*t499.*thetap.*(3.0./4.0)+...
         Io_32.*deltap_o.*t489.*t497.*t500.*thetap.*(3.0./4.0)-Io_33.*deltap_o.*t489.*t496.*t501.*thetap.*(1.0./2.0)-...
         Io_11.*phip_o.*t118.*t211.*t496.*thetap.*(1.0./2.0)-...
         Io_31.*phip_o.*t118.*t207.*t496.*thetap+Io_33.*phip_o.*t118.*t211.*t496.*thetap.*(1.0./2.0)+...
         Io_21.*phip_o.*t118.*t497.*t499.*thetap.*2.0+Io_32.*phip_o.*t118.*t497.*t498.*thetap.*2.0-...
         Io_11.*phip_o.*t211.*t489.*t497.*thetap.*(1.0./2.0)-Io_31.*phip_o.*t207.*t489.*t497.*thetap+...
         Io_33.*phip_o.*t211.*t489.*t497.*thetap.*(1.0./2.0)-Io_21.*phip_o.*t489.*t496.*t499.*thetap.*2.0-...
         Io_32.*phip_o.*t489.*t496.*t498.*thetap.*2.0;
     
    Q81 = f_phi_r-Ir_31.*t4.*t507+Ir_32.*t2.*t4.*t503-Ir_31.*t3.*t4.*t507-Ir_31.*t3.*t4.*t509+Ir_22.*t4.*t504.*t506-Ir_22.*t4.*t504.*t508+...
          Ir_31.*t4.*t503.*t505.*3.0-Ir_31.*t4.*t508.*t509-Ir_31.*t17.*t503.*t506+Ir_31.*t17.*t505.*t506+Ir_22.*phip_r.*t2.*t3.*thetap.*2.0+...
          Ir_21.*phip_r.*t502.*t506.*thetap.*2.0-Ir_21.*phip_r.*t502.*t508.*thetap.*2.0+Ir_32.*phip_r.*t504.*t506.*thetap.*2.0-...
          Ir_32.*phip_r.*t504.*t508.*thetap.*2.0-Ir_32.*t2.*t3.*t4.*t505.*4.0+Ir_21.*t2.*t3.*t17.*t504-Ir_32.*t2.*t3.*t17.*t502+...
          Ir_11.*t3.*t4.*t503.*t504-Ir_21.*t2.*t4.*t502.*t504-Ir_21.*t2.*t4.*t503.*t504.*2.0+Ir_21.*t2.*t4.*t504.*t505-Ir_31.*t3.*t4.*t502.*t503+...
          Ir_32.*t2.*t4.*t502.*t503+Ir_31.*t3.*t4.*t502.*t505-Ir_32.*t2.*t4.*t502.*t505.*2.0+Ir_31.*t3.*t4.*t503.*t505.*6.0-...
          Ir_33.*t3.*t4.*t503.*t504+Ir_11.*t4.*t502.*t503.*t504-Ir_11.*t4.*t502.*t504.*t505-Ir_11.*t4.*t503.*t504.*t506+...
          Ir_11.*t4.*t503.*t504.*t508+Ir_22.*t4.*t502.*t504.*t506+Ir_11.*t17.*t502.*t504.*t506-Ir_33.*t4.*t502.*t503.*t504.*2.0-...
          Ir_31.*t4.*t502.*t505.*t506.*2.0+Ir_31.*t4.*t502.*t505.*t508.*2.0+Ir_31.*t4.*t503.*t505.*t508.*3.0-Ir_33.*t4.*t504.*t505.*t506+...
          Ir_33.*t4.*t504.*t505.*t508-Ir_33.*t17.*t502.*t504.*t506-Ir_11.*phip_r.*t2.*t3.*t503.*thetap.*2.0-Ir_33.*phip_r.*t2.*t3.*t505.*thetap.*2.0-...
          Ir_21.*t2.*t3.*t4.*t502.*t504.*4.0-Ir_21.*t2.*t3.*t4.*t503.*t504.*2.0+Ir_21.*t2.*t3.*t4.*t504.*t505-Ir_32.*t2.*t3.*t4.*t502.*t505.*3.0+...
          Ir_11.*t3.*t4.*t502.*t503.*t504.*2.0-Ir_11.*t3.*t4.*t502.*t504.*t505.*2.0-Ir_33.*t3.*t4.*t502.*t503.*t504.*2.0+Ir_33.*t3.*t4.*t502.*t504.*t505.*2.0+...
          Ir_11.*t4.*t502.*t503.*t504.*t508-Ir_11.*t4.*t502.*t504.*t505.*t508+Ir_33.*t4.*t502.*t504.*t505.*t508.*2.0-Ir_31.*phip_r.*t2.*t3.*t502.*t504.*thetap.*4.0;
     
    Q91 = f_phi_l-Il_31.*t4.*t514+Il_32.*t2.*t4.*t511-Il_31.*t3.*t4.*t514-Il_31.*t3.*t4.*t515+Il_22.*t4.*t506.*t512-Il_22.*t4.*t508.*t512-Il_31.*t4.*t508.*t515+...
          Il_31.*t4.*t511.*t513.*3.0-Il_31.*t15.*t506.*t511+Il_31.*t15.*t506.*t513+Il_22.*phip_l.*t2.*t3.*thetap.*2.0+Il_21.*phip_l.*t506.*t510.*thetap.*2.0-...
          Il_21.*phip_l.*t508.*t510.*thetap.*2.0+Il_32.*phip_l.*t506.*t512.*thetap.*2.0-Il_32.*phip_l.*t508.*t512.*thetap.*2.0+Il_21.*t2.*t3.*t15.*t512-...
          Il_32.*t2.*t3.*t4.*t513.*4.0-Il_32.*t2.*t3.*t15.*t510+Il_11.*t3.*t4.*t511.*t512-Il_21.*t2.*t4.*t510.*t512-Il_21.*t2.*t4.*t511.*t512.*2.0+Il_21.*t2.*t4.*t512.*t513-...
          Il_31.*t3.*t4.*t510.*t511+Il_32.*t2.*t4.*t510.*t511+Il_31.*t3.*t4.*t510.*t513-Il_32.*t2.*t4.*t510.*t513.*2.0+Il_31.*t3.*t4.*t511.*t513.*6.0-Il_33.*t3.*t4.*t511.*t512-...
          Il_11.*t4.*t506.*t511.*t512+Il_11.*t4.*t508.*t511.*t512+Il_11.*t4.*t510.*t511.*t512-Il_11.*t4.*t510.*t512.*t513+Il_11.*t15.*t506.*t510.*t512+Il_22.*t4.*t506.*t510.*t512-...
          Il_31.*t4.*t506.*t510.*t513.*2.0+Il_31.*t4.*t508.*t510.*t513.*2.0+Il_31.*t4.*t508.*t511.*t513.*3.0-Il_33.*t4.*t506.*t512.*t513+Il_33.*t4.*t508.*t512.*t513-...
          Il_33.*t4.*t510.*t511.*t512.*2.0-Il_33.*t15.*t506.*t510.*t512-Il_11.*phip_l.*t2.*t3.*t511.*thetap.*2.0-Il_33.*phip_l.*t2.*t3.*t513.*thetap.*2.0-...
          Il_21.*t2.*t3.*t4.*t510.*t512.*4.0-Il_21.*t2.*t3.*t4.*t511.*t512.*2.0+Il_21.*t2.*t3.*t4.*t512.*t513-Il_32.*t2.*t3.*t4.*t510.*t513.*3.0+Il_11.*t3.*t4.*t510.*t511.*t512.*2.0-...
          Il_11.*t3.*t4.*t510.*t512.*t513.*2.0-Il_33.*t3.*t4.*t510.*t511.*t512.*2.0+Il_33.*t3.*t4.*t510.*t512.*t513.*2.0+Il_11.*t4.*t508.*t510.*t511.*t512-...
          Il_11.*t4.*t508.*t510.*t512.*t513+Il_33.*t4.*t508.*t510.*t512.*t513.*2.0-Il_31.*phip_l.*t2.*t3.*t510.*t512.*thetap.*4.0;
     
     Q = [Q11; Q21; Q31; Q41; Q51; Q61; Q71; Q81; Q91];
